simulink model "ansiOctComp"  (R2018a)
settings: Solver=VariableStepAuto  StartTime=0.0  StopTime=0.001  RelTol=1e-3
undefined symbols (not defined in the file): fdesignblkfcn, G1, G2, G3, G4, G5, G6, G7, G8, gcbh, get, T
libraries: dspsrcs4 x1, dspxfrm3 x1, dspobslib x1
(part 3 of 3)

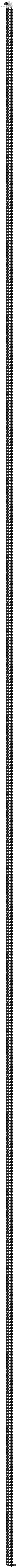
== system ansiOctComp/Filter Bank /Filter 2/Bandpass Filter/Generated Filter Block ==
  Input : Inport
  BodyDelay{2..528} (527 alike) : Delay  DelayLength=1  InitialCondition=0
  BodyLSum{2..528} (527 alike) : Sum  Inputs=++|  RndMeth=Nearest  SaturateOnIntegerOverflow=on  OutDataTypeStr=Inherit: Same as first input
  b(1) : Gain  Gain=0.0013189957886183244  ParamDataTypeStr=double  RndMeth=Nearest  SaturateOnIntegerOverflow=on  OutDataTypeStr=Inherit: Same as input
  b(10) : Gain  Gain=0.000128994813916388394  ParamDataTypeStr=double  RndMeth=Nearest  SaturateOnIntegerOverflow=on  OutDataTypeStr=Inherit: Same as input
  b(100) : Gain  Gain=-0.000423533495409219316  ParamDataTypeStr=double  RndMeth=Nearest  SaturateOnIntegerOverflow=on  OutDataTypeStr=Inherit: Same as input
  b(101) : Gain  Gain=-0.000461669334225578475  ParamDataTypeStr=double  RndMeth=Nearest  SaturateOnIntegerOverflow=on  OutDataTypeStr=Inherit: Same as input
  b(102) : Gain  Gain=-0.000499272274876905349  ParamDataTypeStr=double  RndMeth=Nearest  SaturateOnIntegerOverflow=on  OutDataTypeStr=Inherit: Same as input
  b(103) : Gain  Gain=-0.000536759002049947602  ParamDataTypeStr=double  RndMeth=Nearest  SaturateOnIntegerOverflow=on  OutDataTypeStr=Inherit: Same as input
  b(104) : Gain  Gain=-0.00057288638177031251  ParamDataTypeStr=double  RndMeth=Nearest  SaturateOnIntegerOverflow=on  OutDataTypeStr=Inherit: Same as input
  b(105) : Gain  Gain=-0.000608018296520356112  ParamDataTypeStr=double  RndMeth=Nearest  SaturateOnIntegerOverflow=on  OutDataTypeStr=Inherit: Same as input
  b(106) : Gain  Gain=-0.000640997939764448256  ParamDataTypeStr=double  RndMeth=Nearest  SaturateOnIntegerOverflow=on  OutDataTypeStr=Inherit: Same as input
  b(107) : Gain  Gain=-0.000672143479130331268  ParamDataTypeStr=double  RndMeth=Nearest  SaturateOnIntegerOverflow=on  OutDataTypeStr=Inherit: Same as input
  b(108) : Gain  Gain=-0.000700138237773947664  ParamDataTypeStr=double  RndMeth=Nearest  SaturateOnIntegerOverflow=on  OutDataTypeStr=Inherit: Same as input
  b(109) : Gain  Gain=-0.000725457005707568739  ParamDataTypeStr=double  RndMeth=Nearest  SaturateOnIntegerOverflow=on  OutDataTypeStr=Inherit: Same as input
  b(11) : Gain  Gain=0.000125642526667612978  ParamDataTypeStr=double  RndMeth=Nearest  SaturateOnIntegerOverflow=on  OutDataTypeStr=Inherit: Same as input
  b(110) : Gain  Gain=-0.000746694212294661563  ParamDataTypeStr=double  RndMeth=Nearest  SaturateOnIntegerOverflow=on  OutDataTypeStr=Inherit: Same as input
  b(111) : Gain  Gain=-0.000764284945513389754  ParamDataTypeStr=double  RndMeth=Nearest  SaturateOnIntegerOverflow=on  OutDataTypeStr=Inherit: Same as input
  b(112) : Gain  Gain=-0.000776912328953108179  ParamDataTypeStr=double  RndMeth=Nearest  SaturateOnIntegerOverflow=on  OutDataTypeStr=Inherit: Same as input
  b(113) : Gain  Gain=-0.000784985189046555625  ParamDataTypeStr=double  RndMeth=Nearest  SaturateOnIntegerOverflow=on  OutDataTypeStr=Inherit: Same as input
  b(114) : Gain  Gain=-0.000787233425354552717  ParamDataTypeStr=double  RndMeth=Nearest  SaturateOnIntegerOverflow=on  OutDataTypeStr=Inherit: Same as input
  b(115) : Gain  Gain=-0.00078403753021555095  ParamDataTypeStr=double  RndMeth=Nearest  SaturateOnIntegerOverflow=on  OutDataTypeStr=Inherit: Same as input
  b(116) : Gain  Gain=-0.000774164375811770954  ParamDataTypeStr=double  RndMeth=Nearest  SaturateOnIntegerOverflow=on  OutDataTypeStr=Inherit: Same as input
  b(117) : Gain  Gain=-0.00075805870009854092  ParamDataTypeStr=double  RndMeth=Nearest  SaturateOnIntegerOverflow=on  OutDataTypeStr=Inherit: Same as input
  b(118) : Gain  Gain=-0.000734569828311722726  ParamDataTypeStr=double  RndMeth=Nearest  SaturateOnIntegerOverflow=on  OutDataTypeStr=Inherit: Same as input
  b(119) : Gain  Gain=-0.000704141633403310195  ParamDataTypeStr=double  RndMeth=Nearest  SaturateOnIntegerOverflow=on  OutDataTypeStr=Inherit: Same as input
  b(12) : Gain  Gain=0.000122046249196258033  ParamDataTypeStr=double  RndMeth=Nearest  SaturateOnIntegerOverflow=on  OutDataTypeStr=Inherit: Same as input
  b(120) : Gain  Gain=-0.000665646484304962876  ParamDataTypeStr=double  RndMeth=Nearest  SaturateOnIntegerOverflow=on  OutDataTypeStr=Inherit: Same as input
  b(121) : Gain  Gain=-0.000619640367190464419  ParamDataTypeStr=double  RndMeth=Nearest  SaturateOnIntegerOverflow=on  OutDataTypeStr=Inherit: Same as input
  b(122) : Gain  Gain=-0.000565134472783350244  ParamDataTypeStr=double  RndMeth=Nearest  SaturateOnIntegerOverflow=on  OutDataTypeStr=Inherit: Same as input
  b(123) : Gain  Gain=-0.000502625089221949307  ParamDataTypeStr=double  RndMeth=Nearest  SaturateOnIntegerOverflow=on  OutDataTypeStr=Inherit: Same as input
  b(124) : Gain  Gain=-0.000431307266994649828  ParamDataTypeStr=double  RndMeth=Nearest  SaturateOnIntegerOverflow=on  OutDataTypeStr=Inherit: Same as input
  b(125) : Gain  Gain=-0.000351769691493805832  ParamDataTypeStr=double  RndMeth=Nearest  SaturateOnIntegerOverflow=on  OutDataTypeStr=Inherit: Same as input
  b(126) : Gain  Gain=-0.000263221131644026524  ParamDataTypeStr=double  RndMeth=Nearest  SaturateOnIntegerOverflow=on  OutDataTypeStr=Inherit: Same as input
  b(127) : Gain  Gain=-0.000166409873705706049  ParamDataTypeStr=double  RndMeth=Nearest  SaturateOnIntegerOverflow=on  OutDataTypeStr=Inherit: Same as input
  b(128) : Gain  Gain=-6.06350808818785243e-05  ParamDataTypeStr=double  RndMeth=Nearest  SaturateOnIntegerOverflow=on  OutDataTypeStr=Inherit: Same as input
  b(129) : Gain  Gain=5.3221221105915692e-05  ParamDataTypeStr=double  RndMeth=Nearest  SaturateOnIntegerOverflow=on  OutDataTypeStr=Inherit: Same as input
  b(13) : Gain  Gain=0.000115908705622264248  ParamDataTypeStr=double  RndMeth=Nearest  SaturateOnIntegerOverflow=on  OutDataTypeStr=Inherit: Same as input
  b(130) : Gain  Gain=0.000175769318122429323  ParamDataTypeStr=double  RndMeth=Nearest  SaturateOnIntegerOverflow=on  OutDataTypeStr=Inherit: Same as input
  b(131) : Gain  Gain=0.000306041227612374213  ParamDataTypeStr=double  RndMeth=Nearest  SaturateOnIntegerOverflow=on  OutDataTypeStr=Inherit: Same as input
  b(132) : Gain  Gain=0.000444512367971374497  ParamDataTypeStr=double  RndMeth=Nearest  SaturateOnIntegerOverflow=on  OutDataTypeStr=Inherit: Same as input
  b(133) : Gain  Gain=0.000590057589736560101  ParamDataTypeStr=double  RndMeth=Nearest  SaturateOnIntegerOverflow=on  OutDataTypeStr=Inherit: Same as input
  b(134) : Gain  Gain=0.000743040070891614452  ParamDataTypeStr=double  RndMeth=Nearest  SaturateOnIntegerOverflow=on  OutDataTypeStr=Inherit: Same as input
  b(135) : Gain  Gain=0.000902265678969772192  ParamDataTypeStr=double  RndMeth=Nearest  SaturateOnIntegerOverflow=on  OutDataTypeStr=Inherit: Same as input
  b(136) : Gain  Gain=0.00106797088471714927  ParamDataTypeStr=double  RndMeth=Nearest  SaturateOnIntegerOverflow=on  OutDataTypeStr=Inherit: Same as input
  b(137) : Gain  Gain=0.00123877378306479539  ParamDataTypeStr=double  RndMeth=Nearest  SaturateOnIntegerOverflow=on  OutDataTypeStr=Inherit: Same as input
  b(138) : Gain  Gain=0.00141487218687043554  ParamDataTypeStr=double  RndMeth=Nearest  SaturateOnIntegerOverflow=on  OutDataTypeStr=Inherit: Same as input
  b(139) : Gain  Gain=0.00159476176493942136  ParamDataTypeStr=double  RndMeth=Nearest  SaturateOnIntegerOverflow=on  OutDataTypeStr=Inherit: Same as input
  b(14) : Gain  Gain=0.000109424395758821007  ParamDataTypeStr=double  RndMeth=Nearest  SaturateOnIntegerOverflow=on  OutDataTypeStr=Inherit: Same as input
  b(140) : Gain  Gain=0.00177845198936645564  ParamDataTypeStr=double  RndMeth=Nearest  SaturateOnIntegerOverflow=on  OutDataTypeStr=Inherit: Same as input
  b(141) : Gain  Gain=0.0019644273961855049  ParamDataTypeStr=double  RndMeth=Nearest  SaturateOnIntegerOverflow=on  OutDataTypeStr=Inherit: Same as input
  b(142) : Gain  Gain=0.00215255509300310262  ParamDataTypeStr=double  RndMeth=Nearest  SaturateOnIntegerOverflow=on  OutDataTypeStr=Inherit: Same as input
  b(143) : Gain  Gain=0.00234124102603082635  ParamDataTypeStr=double  RndMeth=Nearest  SaturateOnIntegerOverflow=on  OutDataTypeStr=Inherit: Same as input
  b(144) : Gain  Gain=0.00253023101632903575  ParamDataTypeStr=double  RndMeth=Nearest  SaturateOnIntegerOverflow=on  OutDataTypeStr=Inherit: Same as input
  b(145) : Gain  Gain=0.0027178557454954292  ParamDataTypeStr=double  RndMeth=Nearest  SaturateOnIntegerOverflow=on  OutDataTypeStr=Inherit: Same as input
  b(146) : Gain  Gain=0.00290381159203095124  ParamDataTypeStr=double  RndMeth=Nearest  SaturateOnIntegerOverflow=on  OutDataTypeStr=Inherit: Same as input
  b(147) : Gain  Gain=0.00308638207372412135  ParamDataTypeStr=double  RndMeth=Nearest  SaturateOnIntegerOverflow=on  OutDataTypeStr=Inherit: Same as input
  b(148) : Gain  Gain=0.00326516612697404403  ParamDataTypeStr=double  RndMeth=Nearest  SaturateOnIntegerOverflow=on  OutDataTypeStr=Inherit: Same as input
  b(149) : Gain  Gain=0.00343839387437318202  ParamDataTypeStr=double  RndMeth=Nearest  SaturateOnIntegerOverflow=on  OutDataTypeStr=Inherit: Same as input
  b(15) : Gain  Gain=0.000100118512988072762  ParamDataTypeStr=double  RndMeth=Nearest  SaturateOnIntegerOverflow=on  OutDataTypeStr=Inherit: Same as input
  b(150) : Gain  Gain=0.00360564932851902388  ParamDataTypeStr=double  RndMeth=Nearest  SaturateOnIntegerOverflow=on  OutDataTypeStr=Inherit: Same as input
  b(151) : Gain  Gain=0.00376516794268936172  ParamDataTypeStr=double  RndMeth=Nearest  SaturateOnIntegerOverflow=on  OutDataTypeStr=Inherit: Same as input
  b(152) : Gain  Gain=0.00391645258241414898  ParamDataTypeStr=double  RndMeth=Nearest  SaturateOnIntegerOverflow=on  OutDataTypeStr=Inherit: Same as input
  b(153) : Gain  Gain=0.00405777405273261005  ParamDataTypeStr=double  RndMeth=Nearest  SaturateOnIntegerOverflow=on  OutDataTypeStr=Inherit: Same as input
  b(154) : Gain  Gain=0.00418867978645957092  ParamDataTypeStr=double  RndMeth=Nearest  SaturateOnIntegerOverflow=on  OutDataTypeStr=Inherit: Same as input
  b(155) : Gain  Gain=0.0043073826617828579  ParamDataTypeStr=double  RndMeth=Nearest  SaturateOnIntegerOverflow=on  OutDataTypeStr=Inherit: Same as input
  b(156) : Gain  Gain=0.00441351242527037672  ParamDataTypeStr=double  RndMeth=Nearest  SaturateOnIntegerOverflow=on  OutDataTypeStr=Inherit: Same as input
  b(157) : Gain  Gain=0.00450533688353090857  ParamDataTypeStr=double  RndMeth=Nearest  SaturateOnIntegerOverflow=on  OutDataTypeStr=Inherit: Same as input
  b(158) : Gain  Gain=0.00458254074599091094  ParamDataTypeStr=double  RndMeth=Nearest  SaturateOnIntegerOverflow=on  OutDataTypeStr=Inherit: Same as input
  b(159) : Gain  Gain=0.00464346418155206584  ParamDataTypeStr=double  RndMeth=Nearest  SaturateOnIntegerOverflow=on  OutDataTypeStr=Inherit: Same as input
  b(16) : Gain  Gain=9.42827838523885992e-05  ParamDataTypeStr=double  RndMeth=Nearest  SaturateOnIntegerOverflow=on  OutDataTypeStr=Inherit: Same as input
  b(160) : Gain  Gain=0.00468784260596036978  ParamDataTypeStr=double  RndMeth=Nearest  SaturateOnIntegerOverflow=on  OutDataTypeStr=Inherit: Same as input
  b(161) : Gain  Gain=0.00471414582817185693  ParamDataTypeStr=double  RndMeth=Nearest  SaturateOnIntegerOverflow=on  OutDataTypeStr=Inherit: Same as input
  b(162) : Gain  Gain=0.00472223215326236789  ParamDataTypeStr=double  RndMeth=Nearest  SaturateOnIntegerOverflow=on  OutDataTypeStr=Inherit: Same as input
  b(163) : Gain  Gain=0.00471069265375758696  ParamDataTypeStr=double  RndMeth=Nearest  SaturateOnIntegerOverflow=on  OutDataTypeStr=Inherit: Same as input
  b(164) : Gain  Gain=0.00467948532462431933  ParamDataTypeStr=double  RndMeth=Nearest  SaturateOnIntegerOverflow=on  OutDataTypeStr=Inherit: Same as input
  b(165) : Gain  Gain=0.00462737166796193655  ParamDataTypeStr=double  RndMeth=Nearest  SaturateOnIntegerOverflow=on  OutDataTypeStr=Inherit: Same as input
  b(166) : Gain  Gain=0.00455448397919440591  ParamDataTypeStr=double  RndMeth=Nearest  SaturateOnIntegerOverflow=on  OutDataTypeStr=Inherit: Same as input
  b(167) : Gain  Gain=0.00445973230065942021  ParamDataTypeStr=double  RndMeth=Nearest  SaturateOnIntegerOverflow=on  OutDataTypeStr=Inherit: Same as input
  b(168) : Gain  Gain=0.00434340083942166052  ParamDataTypeStr=double  RndMeth=Nearest  SaturateOnIntegerOverflow=on  OutDataTypeStr=Inherit: Same as input
  b(169) : Gain  Gain=0.00420466577279327014  ParamDataTypeStr=double  RndMeth=Nearest  SaturateOnIntegerOverflow=on  OutDataTypeStr=Inherit: Same as input
  b(17) : Gain  Gain=8.34713962025901597e-05  ParamDataTypeStr=double  RndMeth=Nearest  SaturateOnIntegerOverflow=on  OutDataTypeStr=Inherit: Same as input
  b(170) : Gain  Gain=0.00404392562049606889  ParamDataTypeStr=double  RndMeth=Nearest  SaturateOnIntegerOverflow=on  OutDataTypeStr=Inherit: Same as input
  b(171) : Gain  Gain=0.00386057987620588502  ParamDataTypeStr=double  RndMeth=Nearest  SaturateOnIntegerOverflow=on  OutDataTypeStr=Inherit: Same as input
  b(172) : Gain  Gain=0.00365524307304546667  ParamDataTypeStr=double  RndMeth=Nearest  SaturateOnIntegerOverflow=on  OutDataTypeStr=Inherit: Same as input
  b(173) : Gain  Gain=0.00342754062478000223  ParamDataTypeStr=double  RndMeth=Nearest  SaturateOnIntegerOverflow=on  OutDataTypeStr=Inherit: Same as input
  b(174) : Gain  Gain=0.00317830525562316476  ParamDataTypeStr=double  RndMeth=Nearest  SaturateOnIntegerOverflow=on  OutDataTypeStr=Inherit: Same as input
  b(175) : Gain  Gain=0.00290736343473789721  ParamDataTypeStr=double  RndMeth=Nearest  SaturateOnIntegerOverflow=on  OutDataTypeStr=Inherit: Same as input
  b(176) : Gain  Gain=0.00261576565085099412  ParamDataTypeStr=double  RndMeth=Nearest  SaturateOnIntegerOverflow=on  OutDataTypeStr=Inherit: Same as input
  b(177) : Gain  Gain=0.00230359584321299495  ParamDataTypeStr=double  RndMeth=Nearest  SaturateOnIntegerOverflow=on  OutDataTypeStr=Inherit: Same as input
  b(178) : Gain  Gain=0.00197212374635451606  ParamDataTypeStr=double  RndMeth=Nearest  SaturateOnIntegerOverflow=on  OutDataTypeStr=Inherit: Same as input
  b(179) : Gain  Gain=0.00162164490904748246  ParamDataTypeStr=double  RndMeth=Nearest  SaturateOnIntegerOverflow=on  OutDataTypeStr=Inherit: Same as input
  b(18) : Gain  Gain=7.22562062001517146e-05  ParamDataTypeStr=double  RndMeth=Nearest  SaturateOnIntegerOverflow=on  OutDataTypeStr=Inherit: Same as input
  b(180) : Gain  Gain=0.00125364014383198136  ParamDataTypeStr=double  RndMeth=Nearest  SaturateOnIntegerOverflow=on  OutDataTypeStr=Inherit: Same as input
  b(181) : Gain  Gain=0.000868655989237555122  ParamDataTypeStr=double  RndMeth=Nearest  SaturateOnIntegerOverflow=on  OutDataTypeStr=Inherit: Same as input
  b(182) : Gain  Gain=0.000468370867632063054  ParamDataTypeStr=double  RndMeth=Nearest  SaturateOnIntegerOverflow=on  OutDataTypeStr=Inherit: Same as input
  b(183) : Gain  Gain=5.35140472290680444e-05  ParamDataTypeStr=double  RndMeth=Nearest  SaturateOnIntegerOverflow=on  OutDataTypeStr=Inherit: Same as input
  b(184) : Gain  Gain=-0.000373983290647662229  ParamDataTypeStr=double  RndMeth=Nearest  SaturateOnIntegerOverflow=on  OutDataTypeStr=Inherit: Same as input
  b(185) : Gain  Gain=-0.000813211352745061991  ParamDataTypeStr=double  RndMeth=Nearest  SaturateOnIntegerOverflow=on  OutDataTypeStr=Inherit: Same as input
  b(186) : Gain  Gain=-0.00126209603155125281  ParamDataTypeStr=double  RndMeth=Nearest  SaturateOnIntegerOverflow=on  OutDataTypeStr=Inherit: Same as input
  b(187) : Gain  Gain=-0.0017195185695295912  ParamDataTypeStr=double  RndMeth=Nearest  SaturateOnIntegerOverflow=on  OutDataTypeStr=Inherit: Same as input
  b(188) : Gain  Gain=-0.00218326323704426785  ParamDataTypeStr=double  RndMeth=Nearest  SaturateOnIntegerOverflow=on  OutDataTypeStr=Inherit: Same as input
  b(189) : Gain  Gain=-0.00265202428934371588  ParamDataTypeStr=double  RndMeth=Nearest  SaturateOnIntegerOverflow=on  OutDataTypeStr=Inherit: Same as input
  b(19) : Gain  Gain=6.06151093979667883e-05  ParamDataTypeStr=double  RndMeth=Nearest  SaturateOnIntegerOverflow=on  OutDataTypeStr=Inherit: Same as input
  b(190) : Gain  Gain=-0.00312349066678841922  ParamDataTypeStr=double  RndMeth=Nearest  SaturateOnIntegerOverflow=on  OutDataTypeStr=Inherit: Same as input
  b(191) : Gain  Gain=-0.00359623038932883627  ParamDataTypeStr=double  RndMeth=Nearest  SaturateOnIntegerOverflow=on  OutDataTypeStr=Inherit: Same as input
  b(192) : Gain  Gain=-0.00406783048087909754  ParamDataTypeStr=double  RndMeth=Nearest  SaturateOnIntegerOverflow=on  OutDataTypeStr=Inherit: Same as input
  b(193) : Gain  Gain=-0.00453673939665598207  ParamDataTypeStr=double  RndMeth=Nearest  SaturateOnIntegerOverflow=on  OutDataTypeStr=Inherit: Same as input
  b(194) : Gain  Gain=-0.00500050492305324865  ParamDataTypeStr=double  RndMeth=Nearest  SaturateOnIntegerOverflow=on  OutDataTypeStr=Inherit: Same as input
  b(195) : Gain  Gain=-0.0054575111020349126  ParamDataTypeStr=double  RndMeth=Nearest  SaturateOnIntegerOverflow=on  OutDataTypeStr=Inherit: Same as input
  b(196) : Gain  Gain=-0.00590527600257780439  ParamDataTypeStr=double  RndMeth=Nearest  SaturateOnIntegerOverflow=on  OutDataTypeStr=Inherit: Same as input
  b(197) : Gain  Gain=-0.00634214127357332104  ParamDataTypeStr=double  RndMeth=Nearest  SaturateOnIntegerOverflow=on  OutDataTypeStr=Inherit: Same as input
  b(198) : Gain  Gain=-0.00676568738089359037  ParamDataTypeStr=double  RndMeth=Nearest  SaturateOnIntegerOverflow=on  OutDataTypeStr=Inherit: Same as input
  b(199) : Gain  Gain=-0.00717422804624558326  ParamDataTypeStr=double  RndMeth=Nearest  SaturateOnIntegerOverflow=on  OutDataTypeStr=Inherit: Same as input
  b(2) : Gain  Gain=0.000119600445182501628  ParamDataTypeStr=double  RndMeth=Nearest  SaturateOnIntegerOverflow=on  OutDataTypeStr=Inherit: Same as input
  b(20) : Gain  Gain=4.75559208421214279e-05  ParamDataTypeStr=double  RndMeth=Nearest  SaturateOnIntegerOverflow=on  OutDataTypeStr=Inherit: Same as input
  b(200) : Gain  Gain=-0.00756538283354352657  ParamDataTypeStr=double  RndMeth=Nearest  SaturateOnIntegerOverflow=on  OutDataTypeStr=Inherit: Same as input
  b(201) : Gain  Gain=-0.00793755453304027976  ParamDataTypeStr=double  RndMeth=Nearest  SaturateOnIntegerOverflow=on  OutDataTypeStr=Inherit: Same as input
  b(202) : Gain  Gain=-0.00828844414503448167  ParamDataTypeStr=double  RndMeth=Nearest  SaturateOnIntegerOverflow=on  OutDataTypeStr=Inherit: Same as input
  b(203) : Gain  Gain=-0.00861655179384803772  ParamDataTypeStr=double  RndMeth=Nearest  SaturateOnIntegerOverflow=on  OutDataTypeStr=Inherit: Same as input
  b(204) : Gain  Gain=-0.00891968858251965604  ParamDataTypeStr=double  RndMeth=Nearest  SaturateOnIntegerOverflow=on  OutDataTypeStr=Inherit: Same as input
  b(205) : Gain  Gain=-0.00919649068666273176  ParamDataTypeStr=double  RndMeth=Nearest  SaturateOnIntegerOverflow=on  OutDataTypeStr=Inherit: Same as input
  b(206) : Gain  Gain=-0.00944496004746541058  ParamDataTypeStr=double  RndMeth=Nearest  SaturateOnIntegerOverflow=on  OutDataTypeStr=Inherit: Same as input
  b(207) : Gain  Gain=-0.00966389591080612023  ParamDataTypeStr=double  RndMeth=Nearest  SaturateOnIntegerOverflow=on  OutDataTypeStr=Inherit: Same as input
  b(208) : Gain  Gain=-0.0098514944054812776  ParamDataTypeStr=double  RndMeth=Nearest  SaturateOnIntegerOverflow=on  OutDataTypeStr=Inherit: Same as input
  b(209) : Gain  Gain=-0.010006763264188796  ParamDataTypeStr=double  RndMeth=Nearest  SaturateOnIntegerOverflow=on  OutDataTypeStr=Inherit: Same as input
  b(21) : Gain  Gain=3.35500754738617818e-05  ParamDataTypeStr=double  RndMeth=Nearest  SaturateOnIntegerOverflow=on  OutDataTypeStr=Inherit: Same as input
  b(210) : Gain  Gain=-0.0101281486721101384  ParamDataTypeStr=double  RndMeth=Nearest  SaturateOnIntegerOverflow=on  OutDataTypeStr=Inherit: Same as input
  b(211) : Gain  Gain=-0.0102148848795295486  ParamDataTypeStr=double  RndMeth=Nearest  SaturateOnIntegerOverflow=on  OutDataTypeStr=Inherit: Same as input
  b(212) : Gain  Gain=-0.0102656745807170411  ParamDataTypeStr=double  RndMeth=Nearest  SaturateOnIntegerOverflow=on  OutDataTypeStr=Inherit: Same as input
  b(213) : Gain  Gain=-0.0102800430916763635  ParamDataTypeStr=double  RndMeth=Nearest  SaturateOnIntegerOverflow=on  OutDataTypeStr=Inherit: Same as input
  b(214) : Gain  Gain=-0.0102569951229774387  ParamDataTypeStr=double  RndMeth=Nearest  SaturateOnIntegerOverflow=on  OutDataTypeStr=Inherit: Same as input
  b(215) : Gain  Gain=-0.0101962935444855421  ParamDataTypeStr=double  RndMeth=Nearest  SaturateOnIntegerOverflow=on  OutDataTypeStr=Inherit: Same as input
  b(216) : Gain  Gain=-0.0100972980487470266  ParamDataTypeStr=double  RndMeth=Nearest  SaturateOnIntegerOverflow=on  OutDataTypeStr=Inherit: Same as input
  b(217) : Gain  Gain=-0.00996006829043967305  ParamDataTypeStr=double  RndMeth=Nearest  SaturateOnIntegerOverflow=on  OutDataTypeStr=Inherit: Same as input
  b(218) : Gain  Gain=-0.00978431184645446768  ParamDataTypeStr=double  RndMeth=Nearest  SaturateOnIntegerOverflow=on  OutDataTypeStr=Inherit: Same as input
  b(219) : Gain  Gain=-0.00957038326330438699  ParamDataTypeStr=double  RndMeth=Nearest  SaturateOnIntegerOverflow=on  OutDataTypeStr=Inherit: Same as input
  b(22) : Gain  Gain=1.85707383679374095e-05  ParamDataTypeStr=double  RndMeth=Nearest  SaturateOnIntegerOverflow=on  OutDataTypeStr=Inherit: Same as input
  b(220) : Gain  Gain=-0.00931832776697521722  ParamDataTypeStr=double  RndMeth=Nearest  SaturateOnIntegerOverflow=on  OutDataTypeStr=Inherit: Same as input
  b(221) : Gain  Gain=-0.00902883400440002842  ParamDataTypeStr=double  RndMeth=Nearest  SaturateOnIntegerOverflow=on  OutDataTypeStr=Inherit: Same as input
  b(222) : Gain  Gain=-0.0087022994301005855  ParamDataTypeStr=double  RndMeth=Nearest  SaturateOnIntegerOverflow=on  OutDataTypeStr=Inherit: Same as input
  b(223) : Gain  Gain=-0.00833971895740222291  ParamDataTypeStr=double  RndMeth=Nearest  SaturateOnIntegerOverflow=on  OutDataTypeStr=Inherit: Same as input
  b(224) : Gain  Gain=-0.00794183669351568484  ParamDataTypeStr=double  RndMeth=Nearest  SaturateOnIntegerOverflow=on  OutDataTypeStr=Inherit: Same as input
  b(225) : Gain  Gain=-0.0075099688685431789  ParamDataTypeStr=double  RndMeth=Nearest  SaturateOnIntegerOverflow=on  OutDataTypeStr=Inherit: Same as input
  b(226) : Gain  Gain=-0.00704519052646493914  ParamDataTypeStr=double  RndMeth=Nearest  SaturateOnIntegerOverflow=on  OutDataTypeStr=Inherit: Same as input
  b(227) : Gain  Gain=-0.00654910227540862235  ParamDataTypeStr=double  RndMeth=Nearest  SaturateOnIntegerOverflow=on  OutDataTypeStr=Inherit: Same as input
  b(228) : Gain  Gain=-0.00602310593375914981  ParamDataTypeStr=double  RndMeth=Nearest  SaturateOnIntegerOverflow=on  OutDataTypeStr=Inherit: Same as input
  b(229) : Gain  Gain=-0.00546911525876405454  ParamDataTypeStr=double  RndMeth=Nearest  SaturateOnIntegerOverflow=on  OutDataTypeStr=Inherit: Same as input
  b(23) : Gain  Gain=2.53229324894679517e-06  ParamDataTypeStr=double  RndMeth=Nearest  SaturateOnIntegerOverflow=on  OutDataTypeStr=Inherit: Same as input
  b(230) : Gain  Gain=-0.00488877924777270882  ParamDataTypeStr=double  RndMeth=Nearest  SaturateOnIntegerOverflow=on  OutDataTypeStr=Inherit: Same as input
  b(231) : Gain  Gain=-0.00428427881908863967  ParamDataTypeStr=double  RndMeth=Nearest  SaturateOnIntegerOverflow=on  OutDataTypeStr=Inherit: Same as input
  b(232) : Gain  Gain=-0.00365753396240067925  ParamDataTypeStr=double  RndMeth=Nearest  SaturateOnIntegerOverflow=on  OutDataTypeStr=Inherit: Same as input
  b(233) : Gain  Gain=-0.00301096103934305002  ParamDataTypeStr=double  RndMeth=Nearest  SaturateOnIntegerOverflow=on  OutDataTypeStr=Inherit: Same as input
  b(234) : Gain  Gain=-0.00234670804643675145  ParamDataTypeStr=double  RndMeth=Nearest  SaturateOnIntegerOverflow=on  OutDataTypeStr=Inherit: Same as input
  b(235) : Gain  Gain=-0.0016673640491828871  ParamDataTypeStr=double  RndMeth=Nearest  SaturateOnIntegerOverflow=on  OutDataTypeStr=Inherit: Same as input
  b(236) : Gain  Gain=-0.000975280953428218672  ParamDataTypeStr=double  RndMeth=Nearest  SaturateOnIntegerOverflow=on  OutDataTypeStr=Inherit: Same as input
  b(237) : Gain  Gain=-0.000273203447335550621  ParamDataTypeStr=double  RndMeth=Nearest  SaturateOnIntegerOverflow=on  OutDataTypeStr=Inherit: Same as input
  b(238) : Gain  Gain=0.000436374222012142076  ParamDataTypeStr=double  RndMeth=Nearest  SaturateOnIntegerOverflow=on  OutDataTypeStr=Inherit: Same as input
  b(239) : Gain  Gain=0.00115060614139325798  ParamDataTypeStr=double  RndMeth=Nearest  SaturateOnIntegerOverflow=on  OutDataTypeStr=Inherit: Same as input
  b(24) : Gain  Gain=-1.41991623558972851e-05  ParamDataTypeStr=double  RndMeth=Nearest  SaturateOnIntegerOverflow=on  OutDataTypeStr=Inherit: Same as input
  b(240) : Gain  Gain=0.00186688192354099339  ParamDataTypeStr=double  RndMeth=Nearest  SaturateOnIntegerOverflow=on  OutDataTypeStr=Inherit: Same as input
  b(241) : Gain  Gain=0.0025823010557774642  ParamDataTypeStr=double  RndMeth=Nearest  SaturateOnIntegerOverflow=on  OutDataTypeStr=Inherit: Same as input
  b(242) : Gain  Gain=0.00329420582374038984  ParamDataTypeStr=double  RndMeth=Nearest  SaturateOnIntegerOverflow=on  OutDataTypeStr=Inherit: Same as input
  b(243) : Gain  Gain=0.0039996992447598927  ParamDataTypeStr=double  RndMeth=Nearest  SaturateOnIntegerOverflow=on  OutDataTypeStr=Inherit: Same as input
  b(244) : Gain  Gain=0.00469607268691952899  ParamDataTypeStr=double  RndMeth=Nearest  SaturateOnIntegerOverflow=on  OutDataTypeStr=Inherit: Same as input
  b(245) : Gain  Gain=0.0053804949397835691  ParamDataTypeStr=double  RndMeth=Nearest  SaturateOnIntegerOverflow=on  OutDataTypeStr=Inherit: Same as input
  b(246) : Gain  Gain=0.00605031412425023618  ParamDataTypeStr=double  RndMeth=Nearest  SaturateOnIntegerOverflow=on  OutDataTypeStr=Inherit: Same as input
  b(247) : Gain  Gain=0.00670277986405692482  ParamDataTypeStr=double  RndMeth=Nearest  SaturateOnIntegerOverflow=on  OutDataTypeStr=Inherit: Same as input
  b(248) : Gain  Gain=0.00733532884864761432  ParamDataTypeStr=double  RndMeth=Nearest  SaturateOnIntegerOverflow=on  OutDataTypeStr=Inherit: Same as input
  b(249) : Gain  Gain=0.00794534100781414503  ParamDataTypeStr=double  RndMeth=Nearest  SaturateOnIntegerOverflow=on  OutDataTypeStr=Inherit: Same as input
  b(25) : Gain  Gain=-3.18260172032644104e-05  ParamDataTypeStr=double  RndMeth=Nearest  SaturateOnIntegerOverflow=on  OutDataTypeStr=Inherit: Same as input
  b(250) : Gain  Gain=0.00853041422830583609  ParamDataTypeStr=double  RndMeth=Nearest  SaturateOnIntegerOverflow=on  OutDataTypeStr=Inherit: Same as input
  b(251) : Gain  Gain=0.00908810793177476477  ParamDataTypeStr=double  RndMeth=Nearest  SaturateOnIntegerOverflow=on  OutDataTypeStr=Inherit: Same as input
  b(252) : Gain  Gain=0.0096162011798594238  ParamDataTypeStr=double  RndMeth=Nearest  SaturateOnIntegerOverflow=on  OutDataTypeStr=Inherit: Same as input
  b(253) : Gain  Gain=0.0101124848863965184  ParamDataTypeStr=double  RndMeth=Nearest  SaturateOnIntegerOverflow=on  OutDataTypeStr=Inherit: Same as input
  b(254) : Gain  Gain=0.010574977470715138  ParamDataTypeStr=double  RndMeth=Nearest  SaturateOnIntegerOverflow=on  OutDataTypeStr=Inherit: Same as input
  b(255) : Gain  Gain=0.0110017227247066317  ParamDataTypeStr=double  RndMeth=Nearest  SaturateOnIntegerOverflow=on  OutDataTypeStr=Inherit: Same as input
  b(256) : Gain  Gain=0.0113910099520570553  ParamDataTypeStr=double  RndMeth=Nearest  SaturateOnIntegerOverflow=on  OutDataTypeStr=Inherit: Same as input
  b(257) : Gain  Gain=0.0117411869510578616  ParamDataTypeStr=double  RndMeth=Nearest  SaturateOnIntegerOverflow=on  OutDataTypeStr=Inherit: Same as input
  b(258) : Gain  Gain=0.0120508720478830142  ParamDataTypeStr=double  RndMeth=Nearest  SaturateOnIntegerOverflow=on  OutDataTypeStr=Inherit: Same as input
  b(259) : Gain  Gain=0.0123187129332444495  ParamDataTypeStr=double  RndMeth=Nearest  SaturateOnIntegerOverflow=on  OutDataTypeStr=Inherit: Same as input
  b(26) : Gain  Gain=-4.98086298525179418e-05  ParamDataTypeStr=double  RndMeth=Nearest  SaturateOnIntegerOverflow=on  OutDataTypeStr=Inherit: Same as input
  b(260) : Gain  Gain=0.012543649889335623  ParamDataTypeStr=double  RndMeth=Nearest  SaturateOnIntegerOverflow=on  OutDataTypeStr=Inherit: Same as input
  b(261) : Gain  Gain=0.0127247157071038938  ParamDataTypeStr=double  RndMeth=Nearest  SaturateOnIntegerOverflow=on  OutDataTypeStr=Inherit: Same as input
  b(262) : Gain  Gain=0.0128611926097951038  ParamDataTypeStr=double  RndMeth=Nearest  SaturateOnIntegerOverflow=on  OutDataTypeStr=Inherit: Same as input
  b(263) : Gain  Gain=0.0129524876225628471  ParamDataTypeStr=double  RndMeth=Nearest  SaturateOnIntegerOverflow=on  OutDataTypeStr=Inherit: Same as input
  b(264) : Gain  Gain=0.0129982310171642586  ParamDataTypeStr=double  RndMeth=Nearest  SaturateOnIntegerOverflow=on  OutDataTypeStr=Inherit: Same as input
  b(265) : Gain  Gain=0.0129982310171642586  ParamDataTypeStr=double  RndMeth=Nearest  SaturateOnIntegerOverflow=on  OutDataTypeStr=Inherit: Same as input
  b(266) : Gain  Gain=0.0129524876225628471  ParamDataTypeStr=double  RndMeth=Nearest  SaturateOnIntegerOverflow=on  OutDataTypeStr=Inherit: Same as input
  b(267) : Gain  Gain=0.0128611926097951038  ParamDataTypeStr=double  RndMeth=Nearest  SaturateOnIntegerOverflow=on  OutDataTypeStr=Inherit: Same as input
  b(268) : Gain  Gain=0.0127247157071038938  ParamDataTypeStr=double  RndMeth=Nearest  SaturateOnIntegerOverflow=on  OutDataTypeStr=Inherit: Same as input
  b(269) : Gain  Gain=0.012543649889335623  ParamDataTypeStr=double  RndMeth=Nearest  SaturateOnIntegerOverflow=on  OutDataTypeStr=Inherit: Same as input
  b(27) : Gain  Gain=-6.84426124636459271e-05  ParamDataTypeStr=double  RndMeth=Nearest  SaturateOnIntegerOverflow=on  OutDataTypeStr=Inherit: Same as input
  b(270) : Gain  Gain=0.0123187129332444495  ParamDataTypeStr=double  RndMeth=Nearest  SaturateOnIntegerOverflow=on  OutDataTypeStr=Inherit: Same as input
  b(271) : Gain  Gain=0.0120508720478830142  ParamDataTypeStr=double  RndMeth=Nearest  SaturateOnIntegerOverflow=on  OutDataTypeStr=Inherit: Same as input
  b(272) : Gain  Gain=0.0117411869510578616  ParamDataTypeStr=double  RndMeth=Nearest  SaturateOnIntegerOverflow=on  OutDataTypeStr=Inherit: Same as input
  b(273) : Gain  Gain=0.0113910099520570553  ParamDataTypeStr=double  RndMeth=Nearest  SaturateOnIntegerOverflow=on  OutDataTypeStr=Inherit: Same as input
  b(274) : Gain  Gain=0.0110017227247066317  ParamDataTypeStr=double  RndMeth=Nearest  SaturateOnIntegerOverflow=on  OutDataTypeStr=Inherit: Same as input
  b(275) : Gain  Gain=0.010574977470715138  ParamDataTypeStr=double  RndMeth=Nearest  SaturateOnIntegerOverflow=on  OutDataTypeStr=Inherit: Same as input
  b(276) : Gain  Gain=0.0101124848863965184  ParamDataTypeStr=double  RndMeth=Nearest  SaturateOnIntegerOverflow=on  OutDataTypeStr=Inherit: Same as input
  b(277) : Gain  Gain=0.0096162011798594238  ParamDataTypeStr=double  RndMeth=Nearest  SaturateOnIntegerOverflow=on  OutDataTypeStr=Inherit: Same as input
  b(278) : Gain  Gain=0.00908810793177476477  ParamDataTypeStr=double  RndMeth=Nearest  SaturateOnIntegerOverflow=on  OutDataTypeStr=Inherit: Same as input
  b(279) : Gain  Gain=0.00853041422830583609  ParamDataTypeStr=double  RndMeth=Nearest  SaturateOnIntegerOverflow=on  OutDataTypeStr=Inherit: Same as input
  b(28) : Gain  Gain=-8.73504816807577078e-05  ParamDataTypeStr=double  RndMeth=Nearest  SaturateOnIntegerOverflow=on  OutDataTypeStr=Inherit: Same as input
  b(280) : Gain  Gain=0.00794534100781414503  ParamDataTypeStr=double  RndMeth=Nearest  SaturateOnIntegerOverflow=on  OutDataTypeStr=Inherit: Same as input
  b(281) : Gain  Gain=0.00733532884864761432  ParamDataTypeStr=double  RndMeth=Nearest  SaturateOnIntegerOverflow=on  OutDataTypeStr=Inherit: Same as input
  b(282) : Gain  Gain=0.00670277986405692482  ParamDataTypeStr=double  RndMeth=Nearest  SaturateOnIntegerOverflow=on  OutDataTypeStr=Inherit: Same as input
  b(283) : Gain  Gain=0.00605031412425023618  ParamDataTypeStr=double  RndMeth=Nearest  SaturateOnIntegerOverflow=on  OutDataTypeStr=Inherit: Same as input
  b(284) : Gain  Gain=0.0053804949397835691  ParamDataTypeStr=double  RndMeth=Nearest  SaturateOnIntegerOverflow=on  OutDataTypeStr=Inherit: Same as input
  b(285) : Gain  Gain=0.00469607268691952899  ParamDataTypeStr=double  RndMeth=Nearest  SaturateOnIntegerOverflow=on  OutDataTypeStr=Inherit: Same as input
  b(286) : Gain  Gain=0.0039996992447598927  ParamDataTypeStr=double  RndMeth=Nearest  SaturateOnIntegerOverflow=on  OutDataTypeStr=Inherit: Same as input
  b(287) : Gain  Gain=0.00329420582374038984  ParamDataTypeStr=double  RndMeth=Nearest  SaturateOnIntegerOverflow=on  OutDataTypeStr=Inherit: Same as input
  b(288) : Gain  Gain=0.0025823010557774642  ParamDataTypeStr=double  RndMeth=Nearest  SaturateOnIntegerOverflow=on  OutDataTypeStr=Inherit: Same as input
  b(289) : Gain  Gain=0.00186688192354099339  ParamDataTypeStr=double  RndMeth=Nearest  SaturateOnIntegerOverflow=on  OutDataTypeStr=Inherit: Same as input
  b(29) : Gain  Gain=-0.000106978433770536828  ParamDataTypeStr=double  RndMeth=Nearest  SaturateOnIntegerOverflow=on  OutDataTypeStr=Inherit: Same as input
  b(290) : Gain  Gain=0.00115060614139325798  ParamDataTypeStr=double  RndMeth=Nearest  SaturateOnIntegerOverflow=on  OutDataTypeStr=Inherit: Same as input
  b(291) : Gain  Gain=0.000436374222012142076  ParamDataTypeStr=double  RndMeth=Nearest  SaturateOnIntegerOverflow=on  OutDataTypeStr=Inherit: Same as input
  b(292) : Gain  Gain=-0.000273203447335550621  ParamDataTypeStr=double  RndMeth=Nearest  SaturateOnIntegerOverflow=on  OutDataTypeStr=Inherit: Same as input
  b(293) : Gain  Gain=-0.000975280953428218672  ParamDataTypeStr=double  RndMeth=Nearest  SaturateOnIntegerOverflow=on  OutDataTypeStr=Inherit: Same as input
  b(294) : Gain  Gain=-0.0016673640491828871  ParamDataTypeStr=double  RndMeth=Nearest  SaturateOnIntegerOverflow=on  OutDataTypeStr=Inherit: Same as input
  b(295) : Gain  Gain=-0.00234670804643675145  ParamDataTypeStr=double  RndMeth=Nearest  SaturateOnIntegerOverflow=on  OutDataTypeStr=Inherit: Same as input
  b(296) : Gain  Gain=-0.00301096103934305002  ParamDataTypeStr=double  RndMeth=Nearest  SaturateOnIntegerOverflow=on  OutDataTypeStr=Inherit: Same as input
  b(297) : Gain  Gain=-0.00365753396240067925  ParamDataTypeStr=double  RndMeth=Nearest  SaturateOnIntegerOverflow=on  OutDataTypeStr=Inherit: Same as input
  b(298) : Gain  Gain=-0.00428427881908863967  ParamDataTypeStr=double  RndMeth=Nearest  SaturateOnIntegerOverflow=on  OutDataTypeStr=Inherit: Same as input
  b(299) : Gain  Gain=-0.00488877924777270882  ParamDataTypeStr=double  RndMeth=Nearest  SaturateOnIntegerOverflow=on  OutDataTypeStr=Inherit: Same as input
  b(3) : Gain  Gain=0.000123292979075959085  ParamDataTypeStr=double  RndMeth=Nearest  SaturateOnIntegerOverflow=on  OutDataTypeStr=Inherit: Same as input
  b(30) : Gain  Gain=-0.000127069818868432967  ParamDataTypeStr=double  RndMeth=Nearest  SaturateOnIntegerOverflow=on  OutDataTypeStr=Inherit: Same as input
  b(300) : Gain  Gain=-0.00546911525876405454  ParamDataTypeStr=double  RndMeth=Nearest  SaturateOnIntegerOverflow=on  OutDataTypeStr=Inherit: Same as input
  b(301) : Gain  Gain=-0.00602310593375914981  ParamDataTypeStr=double  RndMeth=Nearest  SaturateOnIntegerOverflow=on  OutDataTypeStr=Inherit: Same as input
  b(302) : Gain  Gain=-0.00654910227540862235  ParamDataTypeStr=double  RndMeth=Nearest  SaturateOnIntegerOverflow=on  OutDataTypeStr=Inherit: Same as input
  b(303) : Gain  Gain=-0.00704519052646493914  ParamDataTypeStr=double  RndMeth=Nearest  SaturateOnIntegerOverflow=on  OutDataTypeStr=Inherit: Same as input
  b(304) : Gain  Gain=-0.0075099688685431789  ParamDataTypeStr=double  RndMeth=Nearest  SaturateOnIntegerOverflow=on  OutDataTypeStr=Inherit: Same as input
  b(305) : Gain  Gain=-0.00794183669351568484  ParamDataTypeStr=double  RndMeth=Nearest  SaturateOnIntegerOverflow=on  OutDataTypeStr=Inherit: Same as input
  b(306) : Gain  Gain=-0.00833971895740222291  ParamDataTypeStr=double  RndMeth=Nearest  SaturateOnIntegerOverflow=on  OutDataTypeStr=Inherit: Same as input
  b(307) : Gain  Gain=-0.0087022994301005855  ParamDataTypeStr=double  RndMeth=Nearest  SaturateOnIntegerOverflow=on  OutDataTypeStr=Inherit: Same as input
  b(308) : Gain  Gain=-0.00902883400440002842  ParamDataTypeStr=double  RndMeth=Nearest  SaturateOnIntegerOverflow=on  OutDataTypeStr=Inherit: Same as input
  b(309) : Gain  Gain=-0.00931832776697521722  ParamDataTypeStr=double  RndMeth=Nearest  SaturateOnIntegerOverflow=on  OutDataTypeStr=Inherit: Same as input
  b(31) : Gain  Gain=-0.000146832212862152119  ParamDataTypeStr=double  RndMeth=Nearest  SaturateOnIntegerOverflow=on  OutDataTypeStr=Inherit: Same as input
  b(310) : Gain  Gain=-0.00957038326330438699  ParamDataTypeStr=double  RndMeth=Nearest  SaturateOnIntegerOverflow=on  OutDataTypeStr=Inherit: Same as input
  b(311) : Gain  Gain=-0.00978431184645446768  ParamDataTypeStr=double  RndMeth=Nearest  SaturateOnIntegerOverflow=on  OutDataTypeStr=Inherit: Same as input
  b(312) : Gain  Gain=-0.00996006829043967305  ParamDataTypeStr=double  RndMeth=Nearest  SaturateOnIntegerOverflow=on  OutDataTypeStr=Inherit: Same as input
  b(313) : Gain  Gain=-0.0100972980487470266  ParamDataTypeStr=double  RndMeth=Nearest  SaturateOnIntegerOverflow=on  OutDataTypeStr=Inherit: Same as input
  b(314) : Gain  Gain=-0.0101962935444855421  ParamDataTypeStr=double  RndMeth=Nearest  SaturateOnIntegerOverflow=on  OutDataTypeStr=Inherit: Same as input
  b(315) : Gain  Gain=-0.0102569951229774387  ParamDataTypeStr=double  RndMeth=Nearest  SaturateOnIntegerOverflow=on  OutDataTypeStr=Inherit: Same as input
  b(316) : Gain  Gain=-0.0102800430916763635  ParamDataTypeStr=double  RndMeth=Nearest  SaturateOnIntegerOverflow=on  OutDataTypeStr=Inherit: Same as input
  b(317) : Gain  Gain=-0.0102656745807170411  ParamDataTypeStr=double  RndMeth=Nearest  SaturateOnIntegerOverflow=on  OutDataTypeStr=Inherit: Same as input
  b(318) : Gain  Gain=-0.0102148848795295486  ParamDataTypeStr=double  RndMeth=Nearest  SaturateOnIntegerOverflow=on  OutDataTypeStr=Inherit: Same as input
  b(319) : Gain  Gain=-0.0101281486721101384  ParamDataTypeStr=double  RndMeth=Nearest  SaturateOnIntegerOverflow=on  OutDataTypeStr=Inherit: Same as input
  b(32) : Gain  Gain=-0.000166417949659631399  ParamDataTypeStr=double  RndMeth=Nearest  SaturateOnIntegerOverflow=on  OutDataTypeStr=Inherit: Same as input
  b(320) : Gain  Gain=-0.010006763264188796  ParamDataTypeStr=double  RndMeth=Nearest  SaturateOnIntegerOverflow=on  OutDataTypeStr=Inherit: Same as input
  b(321) : Gain  Gain=-0.0098514944054812776  ParamDataTypeStr=double  RndMeth=Nearest  SaturateOnIntegerOverflow=on  OutDataTypeStr=Inherit: Same as input
  b(322) : Gain  Gain=-0.00966389591080612023  ParamDataTypeStr=double  RndMeth=Nearest  SaturateOnIntegerOverflow=on  OutDataTypeStr=Inherit: Same as input
  b(323) : Gain  Gain=-0.00944496004746541058  ParamDataTypeStr=double  RndMeth=Nearest  SaturateOnIntegerOverflow=on  OutDataTypeStr=Inherit: Same as input
  b(324) : Gain  Gain=-0.00919649068666273176  ParamDataTypeStr=double  RndMeth=Nearest  SaturateOnIntegerOverflow=on  OutDataTypeStr=Inherit: Same as input
  b(325) : Gain  Gain=-0.00891968858251965604  ParamDataTypeStr=double  RndMeth=Nearest  SaturateOnIntegerOverflow=on  OutDataTypeStr=Inherit: Same as input
  b(326) : Gain  Gain=-0.00861655179384803772  ParamDataTypeStr=double  RndMeth=Nearest  SaturateOnIntegerOverflow=on  OutDataTypeStr=Inherit: Same as input
  b(327) : Gain  Gain=-0.00828844414503448167  ParamDataTypeStr=double  RndMeth=Nearest  SaturateOnIntegerOverflow=on  OutDataTypeStr=Inherit: Same as input
  b(328) : Gain  Gain=-0.00793755453304027976  ParamDataTypeStr=double  RndMeth=Nearest  SaturateOnIntegerOverflow=on  OutDataTypeStr=Inherit: Same as input
  b(329) : Gain  Gain=-0.00756538283354352657  ParamDataTypeStr=double  RndMeth=Nearest  SaturateOnIntegerOverflow=on  OutDataTypeStr=Inherit: Same as input
  b(33) : Gain  Gain=-0.000186903105556324297  ParamDataTypeStr=double  RndMeth=Nearest  SaturateOnIntegerOverflow=on  OutDataTypeStr=Inherit: Same as input
  b(330) : Gain  Gain=-0.00717422804624558326  ParamDataTypeStr=double  RndMeth=Nearest  SaturateOnIntegerOverflow=on  OutDataTypeStr=Inherit: Same as input
  b(331) : Gain  Gain=-0.00676568738089359037  ParamDataTypeStr=double  RndMeth=Nearest  SaturateOnIntegerOverflow=on  OutDataTypeStr=Inherit: Same as input
  b(332) : Gain  Gain=-0.00634214127357332104  ParamDataTypeStr=double  RndMeth=Nearest  SaturateOnIntegerOverflow=on  OutDataTypeStr=Inherit: Same as input
  b(333) : Gain  Gain=-0.00590527600257780439  ParamDataTypeStr=double  RndMeth=Nearest  SaturateOnIntegerOverflow=on  OutDataTypeStr=Inherit: Same as input
  b(334) : Gain  Gain=-0.0054575111020349126  ParamDataTypeStr=double  RndMeth=Nearest  SaturateOnIntegerOverflow=on  OutDataTypeStr=Inherit: Same as input
  b(335) : Gain  Gain=-0.00500050492305324865  ParamDataTypeStr=double  RndMeth=Nearest  SaturateOnIntegerOverflow=on  OutDataTypeStr=Inherit: Same as input
  b(336) : Gain  Gain=-0.00453673939665598207  ParamDataTypeStr=double  RndMeth=Nearest  SaturateOnIntegerOverflow=on  OutDataTypeStr=Inherit: Same as input
  b(337) : Gain  Gain=-0.00406783048087909754  ParamDataTypeStr=double  RndMeth=Nearest  SaturateOnIntegerOverflow=on  OutDataTypeStr=Inherit: Same as input
  b(338) : Gain  Gain=-0.00359623038932883627  ParamDataTypeStr=double  RndMeth=Nearest  SaturateOnIntegerOverflow=on  OutDataTypeStr=Inherit: Same as input
  b(339) : Gain  Gain=-0.00312349066678841922  ParamDataTypeStr=double  RndMeth=Nearest  SaturateOnIntegerOverflow=on  OutDataTypeStr=Inherit: Same as input
  b(34) : Gain  Gain=-0.000206139072550225958  ParamDataTypeStr=double  RndMeth=Nearest  SaturateOnIntegerOverflow=on  OutDataTypeStr=Inherit: Same as input
  b(340) : Gain  Gain=-0.00265202428934371588  ParamDataTypeStr=double  RndMeth=Nearest  SaturateOnIntegerOverflow=on  OutDataTypeStr=Inherit: Same as input
  b(341) : Gain  Gain=-0.00218326323704426785  ParamDataTypeStr=double  RndMeth=Nearest  SaturateOnIntegerOverflow=on  OutDataTypeStr=Inherit: Same as input
  b(342) : Gain  Gain=-0.0017195185695295912  ParamDataTypeStr=double  RndMeth=Nearest  SaturateOnIntegerOverflow=on  OutDataTypeStr=Inherit: Same as input
  b(343) : Gain  Gain=-0.00126209603155125281  ParamDataTypeStr=double  RndMeth=Nearest  SaturateOnIntegerOverflow=on  OutDataTypeStr=Inherit: Same as input
  b(344) : Gain  Gain=-0.000813211352745061991  ParamDataTypeStr=double  RndMeth=Nearest  SaturateOnIntegerOverflow=on  OutDataTypeStr=Inherit: Same as input
  b(345) : Gain  Gain=-0.000373983290647662229  ParamDataTypeStr=double  RndMeth=Nearest  SaturateOnIntegerOverflow=on  OutDataTypeStr=Inherit: Same as input
  b(346) : Gain  Gain=5.35140472290680444e-05  ParamDataTypeStr=double  RndMeth=Nearest  SaturateOnIntegerOverflow=on  OutDataTypeStr=Inherit: Same as input
  b(347) : Gain  Gain=0.000468370867632063054  ParamDataTypeStr=double  RndMeth=Nearest  SaturateOnIntegerOverflow=on  OutDataTypeStr=Inherit: Same as input
  b(348) : Gain  Gain=0.000868655989237555122  ParamDataTypeStr=double  RndMeth=Nearest  SaturateOnIntegerOverflow=on  OutDataTypeStr=Inherit: Same as input
  b(349) : Gain  Gain=0.00125364014383198136  ParamDataTypeStr=double  RndMeth=Nearest  SaturateOnIntegerOverflow=on  OutDataTypeStr=Inherit: Same as input
  b(35) : Gain  Gain=-0.000225875280666558518  ParamDataTypeStr=double  RndMeth=Nearest  SaturateOnIntegerOverflow=on  OutDataTypeStr=Inherit: Same as input
  b(350) : Gain  Gain=0.00162164490904748246  ParamDataTypeStr=double  RndMeth=Nearest  SaturateOnIntegerOverflow=on  OutDataTypeStr=Inherit: Same as input
  b(351) : Gain  Gain=0.00197212374635451606  ParamDataTypeStr=double  RndMeth=Nearest  SaturateOnIntegerOverflow=on  OutDataTypeStr=Inherit: Same as input
  b(352) : Gain  Gain=0.00230359584321299495  ParamDataTypeStr=double  RndMeth=Nearest  SaturateOnIntegerOverflow=on  OutDataTypeStr=Inherit: Same as input
  b(353) : Gain  Gain=0.00261576565085099412  ParamDataTypeStr=double  RndMeth=Nearest  SaturateOnIntegerOverflow=on  OutDataTypeStr=Inherit: Same as input
  b(354) : Gain  Gain=0.00290736343473789721  ParamDataTypeStr=double  RndMeth=Nearest  SaturateOnIntegerOverflow=on  OutDataTypeStr=Inherit: Same as input
  b(355) : Gain  Gain=0.00317830525562316476  ParamDataTypeStr=double  RndMeth=Nearest  SaturateOnIntegerOverflow=on  OutDataTypeStr=Inherit: Same as input
  b(356) : Gain  Gain=0.00342754062478000223  ParamDataTypeStr=double  RndMeth=Nearest  SaturateOnIntegerOverflow=on  OutDataTypeStr=Inherit: Same as input
  b(357) : Gain  Gain=0.00365524307304546667  ParamDataTypeStr=double  RndMeth=Nearest  SaturateOnIntegerOverflow=on  OutDataTypeStr=Inherit: Same as input
  b(358) : Gain  Gain=0.00386057987620588502  ParamDataTypeStr=double  RndMeth=Nearest  SaturateOnIntegerOverflow=on  OutDataTypeStr=Inherit: Same as input
  b(359) : Gain  Gain=0.00404392562049606889  ParamDataTypeStr=double  RndMeth=Nearest  SaturateOnIntegerOverflow=on  OutDataTypeStr=Inherit: Same as input
  b(36) : Gain  Gain=-0.000244422722580023592  ParamDataTypeStr=double  RndMeth=Nearest  SaturateOnIntegerOverflow=on  OutDataTypeStr=Inherit: Same as input
  b(360) : Gain  Gain=0.00420466577279327014  ParamDataTypeStr=double  RndMeth=Nearest  SaturateOnIntegerOverflow=on  OutDataTypeStr=Inherit: Same as input
  b(361) : Gain  Gain=0.00434340083942166052  ParamDataTypeStr=double  RndMeth=Nearest  SaturateOnIntegerOverflow=on  OutDataTypeStr=Inherit: Same as input
  b(362) : Gain  Gain=0.00445973230065942021  ParamDataTypeStr=double  RndMeth=Nearest  SaturateOnIntegerOverflow=on  OutDataTypeStr=Inherit: Same as input
  b(363) : Gain  Gain=0.00455448397919440591  ParamDataTypeStr=double  RndMeth=Nearest  SaturateOnIntegerOverflow=on  OutDataTypeStr=Inherit: Same as input
  b(364) : Gain  Gain=0.00462737166796193655  ParamDataTypeStr=double  RndMeth=Nearest  SaturateOnIntegerOverflow=on  OutDataTypeStr=Inherit: Same as input
  b(365) : Gain  Gain=0.00467948532462431933  ParamDataTypeStr=double  RndMeth=Nearest  SaturateOnIntegerOverflow=on  OutDataTypeStr=Inherit: Same as input
  b(366) : Gain  Gain=0.00471069265375758696  ParamDataTypeStr=double  RndMeth=Nearest  SaturateOnIntegerOverflow=on  OutDataTypeStr=Inherit: Same as input
  b(367) : Gain  Gain=0.00472223215326236789  ParamDataTypeStr=double  RndMeth=Nearest  SaturateOnIntegerOverflow=on  OutDataTypeStr=Inherit: Same as input
  b(368) : Gain  Gain=0.00471414582817185693  ParamDataTypeStr=double  RndMeth=Nearest  SaturateOnIntegerOverflow=on  OutDataTypeStr=Inherit: Same as input
  b(369) : Gain  Gain=0.00468784260596036978  ParamDataTypeStr=double  RndMeth=Nearest  SaturateOnIntegerOverflow=on  OutDataTypeStr=Inherit: Same as input
  b(37) : Gain  Gain=-0.000263040701395831364  ParamDataTypeStr=double  RndMeth=Nearest  SaturateOnIntegerOverflow=on  OutDataTypeStr=Inherit: Same as input
  b(370) : Gain  Gain=0.00464346418155206584  ParamDataTypeStr=double  RndMeth=Nearest  SaturateOnIntegerOverflow=on  OutDataTypeStr=Inherit: Same as input
  b(371) : Gain  Gain=0.00458254074599091094  ParamDataTypeStr=double  RndMeth=Nearest  SaturateOnIntegerOverflow=on  OutDataTypeStr=Inherit: Same as input
  b(372) : Gain  Gain=0.00450533688353090857  ParamDataTypeStr=double  RndMeth=Nearest  SaturateOnIntegerOverflow=on  OutDataTypeStr=Inherit: Same as input
  b(373) : Gain  Gain=0.00441351242527037672  ParamDataTypeStr=double  RndMeth=Nearest  SaturateOnIntegerOverflow=on  OutDataTypeStr=Inherit: Same as input
  b(374) : Gain  Gain=0.0043073826617828579  ParamDataTypeStr=double  RndMeth=Nearest  SaturateOnIntegerOverflow=on  OutDataTypeStr=Inherit: Same as input
  b(375) : Gain  Gain=0.00418867978645957092  ParamDataTypeStr=double  RndMeth=Nearest  SaturateOnIntegerOverflow=on  OutDataTypeStr=Inherit: Same as input
  b(376) : Gain  Gain=0.00405777405273261005  ParamDataTypeStr=double  RndMeth=Nearest  SaturateOnIntegerOverflow=on  OutDataTypeStr=Inherit: Same as input
  b(377) : Gain  Gain=0.00391645258241414898  ParamDataTypeStr=double  RndMeth=Nearest  SaturateOnIntegerOverflow=on  OutDataTypeStr=Inherit: Same as input
  b(378) : Gain  Gain=0.00376516794268936172  ParamDataTypeStr=double  RndMeth=Nearest  SaturateOnIntegerOverflow=on  OutDataTypeStr=Inherit: Same as input
  b(379) : Gain  Gain=0.00360564932851902388  ParamDataTypeStr=double  RndMeth=Nearest  SaturateOnIntegerOverflow=on  OutDataTypeStr=Inherit: Same as input
  b(38) : Gain  Gain=-0.000280358987114503935  ParamDataTypeStr=double  RndMeth=Nearest  SaturateOnIntegerOverflow=on  OutDataTypeStr=Inherit: Same as input
  b(380) : Gain  Gain=0.00343839387437318202  ParamDataTypeStr=double  RndMeth=Nearest  SaturateOnIntegerOverflow=on  OutDataTypeStr=Inherit: Same as input
  b(381) : Gain  Gain=0.00326516612697404403  ParamDataTypeStr=double  RndMeth=Nearest  SaturateOnIntegerOverflow=on  OutDataTypeStr=Inherit: Same as input
  b(382) : Gain  Gain=0.00308638207372412135  ParamDataTypeStr=double  RndMeth=Nearest  SaturateOnIntegerOverflow=on  OutDataTypeStr=Inherit: Same as input
  b(383) : Gain  Gain=0.00290381159203095124  ParamDataTypeStr=double  RndMeth=Nearest  SaturateOnIntegerOverflow=on  OutDataTypeStr=Inherit: Same as input
  b(384) : Gain  Gain=0.0027178557454954292  ParamDataTypeStr=double  RndMeth=Nearest  SaturateOnIntegerOverflow=on  OutDataTypeStr=Inherit: Same as input
  b(385) : Gain  Gain=0.00253023101632903575  ParamDataTypeStr=double  RndMeth=Nearest  SaturateOnIntegerOverflow=on  OutDataTypeStr=Inherit: Same as input
  b(386) : Gain  Gain=0.00234124102603082635  ParamDataTypeStr=double  RndMeth=Nearest  SaturateOnIntegerOverflow=on  OutDataTypeStr=Inherit: Same as input
  b(387) : Gain  Gain=0.00215255509300310262  ParamDataTypeStr=double  RndMeth=Nearest  SaturateOnIntegerOverflow=on  OutDataTypeStr=Inherit: Same as input
  b(388) : Gain  Gain=0.0019644273961855049  ParamDataTypeStr=double  RndMeth=Nearest  SaturateOnIntegerOverflow=on  OutDataTypeStr=Inherit: Same as input
  b(389) : Gain  Gain=0.00177845198936645564  ParamDataTypeStr=double  RndMeth=Nearest  SaturateOnIntegerOverflow=on  OutDataTypeStr=Inherit: Same as input
  b(39) : Gain  Gain=-0.000297528049151355107  ParamDataTypeStr=double  RndMeth=Nearest  SaturateOnIntegerOverflow=on  OutDataTypeStr=Inherit: Same as input
  b(390) : Gain  Gain=0.00159476176493942136  ParamDataTypeStr=double  RndMeth=Nearest  SaturateOnIntegerOverflow=on  OutDataTypeStr=Inherit: Same as input
  b(391) : Gain  Gain=0.00141487218687043554  ParamDataTypeStr=double  RndMeth=Nearest  SaturateOnIntegerOverflow=on  OutDataTypeStr=Inherit: Same as input
  b(392) : Gain  Gain=0.00123877378306479539  ParamDataTypeStr=double  RndMeth=Nearest  SaturateOnIntegerOverflow=on  OutDataTypeStr=Inherit: Same as input
  b(393) : Gain  Gain=0.00106797088471714927  ParamDataTypeStr=double  RndMeth=Nearest  SaturateOnIntegerOverflow=on  OutDataTypeStr=Inherit: Same as input
  b(394) : Gain  Gain=0.000902265678969772192  ParamDataTypeStr=double  RndMeth=Nearest  SaturateOnIntegerOverflow=on  OutDataTypeStr=Inherit: Same as input
  b(395) : Gain  Gain=0.000743040070891614452  ParamDataTypeStr=double  RndMeth=Nearest  SaturateOnIntegerOverflow=on  OutDataTypeStr=Inherit: Same as input
  b(396) : Gain  Gain=0.000590057589736560101  ParamDataTypeStr=double  RndMeth=Nearest  SaturateOnIntegerOverflow=on  OutDataTypeStr=Inherit: Same as input
  b(397) : Gain  Gain=0.000444512367971374497  ParamDataTypeStr=double  RndMeth=Nearest  SaturateOnIntegerOverflow=on  OutDataTypeStr=Inherit: Same as input
  b(398) : Gain  Gain=0.000306041227612374213  ParamDataTypeStr=double  RndMeth=Nearest  SaturateOnIntegerOverflow=on  OutDataTypeStr=Inherit: Same as input
  b(399) : Gain  Gain=0.000175769318122429323  ParamDataTypeStr=double  RndMeth=Nearest  SaturateOnIntegerOverflow=on  OutDataTypeStr=Inherit: Same as input
  b(4) : Gain  Gain=0.000126958318748944705  ParamDataTypeStr=double  RndMeth=Nearest  SaturateOnIntegerOverflow=on  OutDataTypeStr=Inherit: Same as input
  b(40) : Gain  Gain=-0.000313246594477974757  ParamDataTypeStr=double  RndMeth=Nearest  SaturateOnIntegerOverflow=on  OutDataTypeStr=Inherit: Same as input
  b(400) : Gain  Gain=5.3221221105915692e-05  ParamDataTypeStr=double  RndMeth=Nearest  SaturateOnIntegerOverflow=on  OutDataTypeStr=Inherit: Same as input
  b(401) : Gain  Gain=-6.06350808818785243e-05  ParamDataTypeStr=double  RndMeth=Nearest  SaturateOnIntegerOverflow=on  OutDataTypeStr=Inherit: Same as input
  b(402) : Gain  Gain=-0.000166409873705706049  ParamDataTypeStr=double  RndMeth=Nearest  SaturateOnIntegerOverflow=on  OutDataTypeStr=Inherit: Same as input
  b(403) : Gain  Gain=-0.000263221131644026524  ParamDataTypeStr=double  RndMeth=Nearest  SaturateOnIntegerOverflow=on  OutDataTypeStr=Inherit: Same as input
  b(404) : Gain  Gain=-0.000351769691493805832  ParamDataTypeStr=double  RndMeth=Nearest  SaturateOnIntegerOverflow=on  OutDataTypeStr=Inherit: Same as input
  b(405) : Gain  Gain=-0.000431307266994649828  ParamDataTypeStr=double  RndMeth=Nearest  SaturateOnIntegerOverflow=on  OutDataTypeStr=Inherit: Same as input
  b(406) : Gain  Gain=-0.000502625089221949307  ParamDataTypeStr=double  RndMeth=Nearest  SaturateOnIntegerOverflow=on  OutDataTypeStr=Inherit: Same as input
  b(407) : Gain  Gain=-0.000565134472783350244  ParamDataTypeStr=double  RndMeth=Nearest  SaturateOnIntegerOverflow=on  OutDataTypeStr=Inherit: Same as input
  b(408) : Gain  Gain=-0.000619640367190464419  ParamDataTypeStr=double  RndMeth=Nearest  SaturateOnIntegerOverflow=on  OutDataTypeStr=Inherit: Same as input
  b(409) : Gain  Gain=-0.000665646484304962876  ParamDataTypeStr=double  RndMeth=Nearest  SaturateOnIntegerOverflow=on  OutDataTypeStr=Inherit: Same as input
  b(41) : Gain  Gain=-0.000328550564974419397  ParamDataTypeStr=double  RndMeth=Nearest  SaturateOnIntegerOverflow=on  OutDataTypeStr=Inherit: Same as input
  b(410) : Gain  Gain=-0.000704141633403310195  ParamDataTypeStr=double  RndMeth=Nearest  SaturateOnIntegerOverflow=on  OutDataTypeStr=Inherit: Same as input
  b(411) : Gain  Gain=-0.000734569828311722726  ParamDataTypeStr=double  RndMeth=Nearest  SaturateOnIntegerOverflow=on  OutDataTypeStr=Inherit: Same as input
  b(412) : Gain  Gain=-0.00075805870009854092  ParamDataTypeStr=double  RndMeth=Nearest  SaturateOnIntegerOverflow=on  OutDataTypeStr=Inherit: Same as input
  b(413) : Gain  Gain=-0.000774164375811770954  ParamDataTypeStr=double  RndMeth=Nearest  SaturateOnIntegerOverflow=on  OutDataTypeStr=Inherit: Same as input
  b(414) : Gain  Gain=-0.00078403753021555095  ParamDataTypeStr=double  RndMeth=Nearest  SaturateOnIntegerOverflow=on  OutDataTypeStr=Inherit: Same as input
  b(415) : Gain  Gain=-0.000787233425354552717  ParamDataTypeStr=double  RndMeth=Nearest  SaturateOnIntegerOverflow=on  OutDataTypeStr=Inherit: Same as input
  b(416) : Gain  Gain=-0.000784985189046555625  ParamDataTypeStr=double  RndMeth=Nearest  SaturateOnIntegerOverflow=on  OutDataTypeStr=Inherit: Same as input
  b(417) : Gain  Gain=-0.000776912328953108179  ParamDataTypeStr=double  RndMeth=Nearest  SaturateOnIntegerOverflow=on  OutDataTypeStr=Inherit: Same as input
  b(418) : Gain  Gain=-0.000764284945513389754  ParamDataTypeStr=double  RndMeth=Nearest  SaturateOnIntegerOverflow=on  OutDataTypeStr=Inherit: Same as input
  b(419) : Gain  Gain=-0.000746694212294661563  ParamDataTypeStr=double  RndMeth=Nearest  SaturateOnIntegerOverflow=on  OutDataTypeStr=Inherit: Same as input
  b(42) : Gain  Gain=-0.000342087513098722614  ParamDataTypeStr=double  RndMeth=Nearest  SaturateOnIntegerOverflow=on  OutDataTypeStr=Inherit: Same as input
  b(420) : Gain  Gain=-0.000725457005707568739  ParamDataTypeStr=double  RndMeth=Nearest  SaturateOnIntegerOverflow=on  OutDataTypeStr=Inherit: Same as input
  b(421) : Gain  Gain=-0.000700138237773947664  ParamDataTypeStr=double  RndMeth=Nearest  SaturateOnIntegerOverflow=on  OutDataTypeStr=Inherit: Same as input
  b(422) : Gain  Gain=-0.000672143479130331268  ParamDataTypeStr=double  RndMeth=Nearest  SaturateOnIntegerOverflow=on  OutDataTypeStr=Inherit: Same as input
  b(423) : Gain  Gain=-0.000640997939764448256  ParamDataTypeStr=double  RndMeth=Nearest  SaturateOnIntegerOverflow=on  OutDataTypeStr=Inherit: Same as input
  b(424) : Gain  Gain=-0.000608018296520356112  ParamDataTypeStr=double  RndMeth=Nearest  SaturateOnIntegerOverflow=on  OutDataTypeStr=Inherit: Same as input
  b(425) : Gain  Gain=-0.00057288638177031251  ParamDataTypeStr=double  RndMeth=Nearest  SaturateOnIntegerOverflow=on  OutDataTypeStr=Inherit: Same as input
  b(426) : Gain  Gain=-0.000536759002049947602  ParamDataTypeStr=double  RndMeth=Nearest  SaturateOnIntegerOverflow=on  OutDataTypeStr=Inherit: Same as input
  b(427) : Gain  Gain=-0.000499272274876905349  ParamDataTypeStr=double  RndMeth=Nearest  SaturateOnIntegerOverflow=on  OutDataTypeStr=Inherit: Same as input
  b(428) : Gain  Gain=-0.000461669334225578475  ParamDataTypeStr=double  RndMeth=Nearest  SaturateOnIntegerOverflow=on  OutDataTypeStr=Inherit: Same as input
  b(429) : Gain  Gain=-0.000423533495409219316  ParamDataTypeStr=double  RndMeth=Nearest  SaturateOnIntegerOverflow=on  OutDataTypeStr=Inherit: Same as input
  b(43) : Gain  Gain=-0.000354911467429252061  ParamDataTypeStr=double  RndMeth=Nearest  SaturateOnIntegerOverflow=on  OutDataTypeStr=Inherit: Same as input
  b(430) : Gain  Gain=-0.000386007594417995138  ParamDataTypeStr=double  RndMeth=Nearest  SaturateOnIntegerOverflow=on  OutDataTypeStr=Inherit: Same as input
  b(431) : Gain  Gain=-0.000348624240333695939  ParamDataTypeStr=double  RndMeth=Nearest  SaturateOnIntegerOverflow=on  OutDataTypeStr=Inherit: Same as input
  b(432) : Gain  Gain=-0.000312529436229563081  ParamDataTypeStr=double  RndMeth=Nearest  SaturateOnIntegerOverflow=on  OutDataTypeStr=Inherit: Same as input
  b(433) : Gain  Gain=-0.00027723555258353798  ParamDataTypeStr=double  RndMeth=Nearest  SaturateOnIntegerOverflow=on  OutDataTypeStr=Inherit: Same as input
  b(434) : Gain  Gain=-0.000243803841427045562  ParamDataTypeStr=double  RndMeth=Nearest  SaturateOnIntegerOverflow=on  OutDataTypeStr=Inherit: Same as input
  b(435) : Gain  Gain=-0.000211695078287365548  ParamDataTypeStr=double  RndMeth=Nearest  SaturateOnIntegerOverflow=on  OutDataTypeStr=Inherit: Same as input
  b(436) : Gain  Gain=-0.00018187967171705505  ParamDataTypeStr=double  RndMeth=Nearest  SaturateOnIntegerOverflow=on  OutDataTypeStr=Inherit: Same as input
  b(437) : Gain  Gain=-0.000153800533059332729  ParamDataTypeStr=double  RndMeth=Nearest  SaturateOnIntegerOverflow=on  OutDataTypeStr=Inherit: Same as input
  b(438) : Gain  Gain=-0.00012844573614923015  ParamDataTypeStr=double  RndMeth=Nearest  SaturateOnIntegerOverflow=on  OutDataTypeStr=Inherit: Same as input
  b(439) : Gain  Gain=-0.000104999200466021321  ParamDataTypeStr=double  RndMeth=Nearest  SaturateOnIntegerOverflow=on  OutDataTypeStr=Inherit: Same as input
  b(44) : Gain  Gain=-0.000365845398302402621  ParamDataTypeStr=double  RndMeth=Nearest  SaturateOnIntegerOverflow=on  OutDataTypeStr=Inherit: Same as input
  b(440) : Gain  Gain=-8.46336706624266095e-05  ParamDataTypeStr=double  RndMeth=Nearest  SaturateOnIntegerOverflow=on  OutDataTypeStr=Inherit: Same as input
  b(441) : Gain  Gain=-6.63999170443811595e-05  ParamDataTypeStr=double  RndMeth=Nearest  SaturateOnIntegerOverflow=on  OutDataTypeStr=Inherit: Same as input
  b(442) : Gain  Gain=-5.127065973762235e-05  ParamDataTypeStr=double  RndMeth=Nearest  SaturateOnIntegerOverflow=on  OutDataTypeStr=Inherit: Same as input
  b(443) : Gain  Gain=-3.83862678230118774e-05  ParamDataTypeStr=double  RndMeth=Nearest  SaturateOnIntegerOverflow=on  OutDataTypeStr=Inherit: Same as input
  b(444) : Gain  Gain=-2.87166278037361087e-05  ParamDataTypeStr=double  RndMeth=Nearest  SaturateOnIntegerOverflow=on  OutDataTypeStr=Inherit: Same as input
  b(445) : Gain  Gain=-2.12850613980476808e-05  ParamDataTypeStr=double  RndMeth=Nearest  SaturateOnIntegerOverflow=on  OutDataTypeStr=Inherit: Same as input
  b(446) : Gain  Gain=-1.69628308546508448e-05  ParamDataTypeStr=double  RndMeth=Nearest  SaturateOnIntegerOverflow=on  OutDataTypeStr=Inherit: Same as input
  b(447) : Gain  Gain=-1.47437363230819383e-05  ParamDataTypeStr=double  RndMeth=Nearest  SaturateOnIntegerOverflow=on  OutDataTypeStr=Inherit: Same as input
  b(448) : Gain  Gain=-1.55128158049954671e-05  ParamDataTypeStr=double  RndMeth=Nearest  SaturateOnIntegerOverflow=on  OutDataTypeStr=Inherit: Same as input
  b(449) : Gain  Gain=-1.82129216426999644e-05  ParamDataTypeStr=double  RndMeth=Nearest  SaturateOnIntegerOverflow=on  OutDataTypeStr=Inherit: Same as input
  b(45) : Gain  Gain=-0.000376157350598188729  ParamDataTypeStr=double  RndMeth=Nearest  SaturateOnIntegerOverflow=on  OutDataTypeStr=Inherit: Same as input
  b(450) : Gain  Gain=-2.36957211731823793e-05  ParamDataTypeStr=double  RndMeth=Nearest  SaturateOnIntegerOverflow=on  OutDataTypeStr=Inherit: Same as input
  b(451) : Gain  Gain=-3.08383793457291371e-05  ParamDataTypeStr=double  RndMeth=Nearest  SaturateOnIntegerOverflow=on  OutDataTypeStr=Inherit: Same as input
  b(452) : Gain  Gain=-4.04269010002347978e-05  ParamDataTypeStr=double  RndMeth=Nearest  SaturateOnIntegerOverflow=on  OutDataTypeStr=Inherit: Same as input
  b(453) : Gain  Gain=-5.15015329802558704e-05  ParamDataTypeStr=double  RndMeth=Nearest  SaturateOnIntegerOverflow=on  OutDataTypeStr=Inherit: Same as input
  b(454) : Gain  Gain=-6.45312083203074521e-05  ParamDataTypeStr=double  RndMeth=Nearest  SaturateOnIntegerOverflow=on  OutDataTypeStr=Inherit: Same as input
  b(455) : Gain  Gain=-7.87286212535760581e-05  ParamDataTypeStr=double  RndMeth=Nearest  SaturateOnIntegerOverflow=on  OutDataTypeStr=Inherit: Same as input
  b(456) : Gain  Gain=-9.46829036739340896e-05  ParamDataTypeStr=double  RndMeth=Nearest  SaturateOnIntegerOverflow=on  OutDataTypeStr=Inherit: Same as input
  b(457) : Gain  Gain=-0.00011125252133578384  ParamDataTypeStr=double  RndMeth=Nearest  SaturateOnIntegerOverflow=on  OutDataTypeStr=Inherit: Same as input
  b(458) : Gain  Gain=-0.000129141873349178935  ParamDataTypeStr=double  RndMeth=Nearest  SaturateOnIntegerOverflow=on  OutDataTypeStr=Inherit: Same as input
  b(459) : Gain  Gain=-0.000147315132967771201  ParamDataTypeStr=double  RndMeth=Nearest  SaturateOnIntegerOverflow=on  OutDataTypeStr=Inherit: Same as input
  b(46) : Gain  Gain=-0.000384291427222763172  ParamDataTypeStr=double  RndMeth=Nearest  SaturateOnIntegerOverflow=on  OutDataTypeStr=Inherit: Same as input
  b(460) : Gain  Gain=-0.000166478229983800735  ParamDataTypeStr=double  RndMeth=Nearest  SaturateOnIntegerOverflow=on  OutDataTypeStr=Inherit: Same as input
  b(461) : Gain  Gain=-0.000185503270808741157  ParamDataTypeStr=double  RndMeth=Nearest  SaturateOnIntegerOverflow=on  OutDataTypeStr=Inherit: Same as input
  b(462) : Gain  Gain=-0.00020509011935799723  ParamDataTypeStr=double  RndMeth=Nearest  SaturateOnIntegerOverflow=on  OutDataTypeStr=Inherit: Same as input
  b(463) : Gain  Gain=-0.00022414279328602355  ParamDataTypeStr=double  RndMeth=Nearest  SaturateOnIntegerOverflow=on  OutDataTypeStr=Inherit: Same as input
  b(464) : Gain  Gain=-0.000243411438438570623  ParamDataTypeStr=double  RndMeth=Nearest  SaturateOnIntegerOverflow=on  OutDataTypeStr=Inherit: Same as input
  b(465) : Gain  Gain=-0.000261789142866730284  ParamDataTypeStr=double  RndMeth=Nearest  SaturateOnIntegerOverflow=on  OutDataTypeStr=Inherit: Same as input
  b(466) : Gain  Gain=-0.000280071574432796044  ParamDataTypeStr=double  RndMeth=Nearest  SaturateOnIntegerOverflow=on  OutDataTypeStr=Inherit: Same as input
  b(467) : Gain  Gain=-0.000296990192063201945  ParamDataTypeStr=double  RndMeth=Nearest  SaturateOnIntegerOverflow=on  OutDataTypeStr=Inherit: Same as input
  b(468) : Gain  Gain=-0.000313697423958395668  ParamDataTypeStr=double  RndMeth=Nearest  SaturateOnIntegerOverflow=on  OutDataTypeStr=Inherit: Same as input
  b(469) : Gain  Gain=-0.000328612037461096336  ParamDataTypeStr=double  RndMeth=Nearest  SaturateOnIntegerOverflow=on  OutDataTypeStr=Inherit: Same as input
  b(47) : Gain  Gain=-0.000391134875770449662  ParamDataTypeStr=double  RndMeth=Nearest  SaturateOnIntegerOverflow=on  OutDataTypeStr=Inherit: Same as input
  b(470) : Gain  Gain=-0.000342894954706609613  ParamDataTypeStr=double  RndMeth=Nearest  SaturateOnIntegerOverflow=on  OutDataTypeStr=Inherit: Same as input
  b(471) : Gain  Gain=-0.000355511706333689866  ParamDataTypeStr=double  RndMeth=Nearest  SaturateOnIntegerOverflow=on  OutDataTypeStr=Inherit: Same as input
  b(472) : Gain  Gain=-0.000367171401728139373  ParamDataTypeStr=double  RndMeth=Nearest  SaturateOnIntegerOverflow=on  OutDataTypeStr=Inherit: Same as input
  b(473) : Gain  Gain=-0.000376818546642253716  ParamDataTypeStr=double  RndMeth=Nearest  SaturateOnIntegerOverflow=on  OutDataTypeStr=Inherit: Same as input
  b(474) : Gain  Gain=-0.000385359957846202793  ParamDataTypeStr=double  RndMeth=Nearest  SaturateOnIntegerOverflow=on  OutDataTypeStr=Inherit: Same as input
  b(475) : Gain  Gain=-0.000391841892495430836  ParamDataTypeStr=double  RndMeth=Nearest  SaturateOnIntegerOverflow=on  OutDataTypeStr=Inherit: Same as input
  b(476) : Gain  Gain=-0.000397125758577358606  ParamDataTypeStr=double  RndMeth=Nearest  SaturateOnIntegerOverflow=on  OutDataTypeStr=Inherit: Same as input
  b(477) : Gain  Gain=-0.00040023311630166215  ParamDataTypeStr=double  RndMeth=Nearest  SaturateOnIntegerOverflow=on  OutDataTypeStr=Inherit: Same as input
  b(478) : Gain  Gain=-0.000402035792474276111  ParamDataTypeStr=double  RndMeth=Nearest  SaturateOnIntegerOverflow=on  OutDataTypeStr=Inherit: Same as input
  b(479) : Gain  Gain=-0.000401659938941869958  ParamDataTypeStr=double  RndMeth=Nearest  SaturateOnIntegerOverflow=on  OutDataTypeStr=Inherit: Same as input
  b(48) : Gain  Gain=-0.000396279890881591403  ParamDataTypeStr=double  RndMeth=Nearest  SaturateOnIntegerOverflow=on  OutDataTypeStr=Inherit: Same as input
  b(480) : Gain  Gain=-0.000399976844345353204  ParamDataTypeStr=double  RndMeth=Nearest  SaturateOnIntegerOverflow=on  OutDataTypeStr=Inherit: Same as input
  b(481) : Gain  Gain=-0.000396279890881591403  ParamDataTypeStr=double  RndMeth=Nearest  SaturateOnIntegerOverflow=on  OutDataTypeStr=Inherit: Same as input
  b(482) : Gain  Gain=-0.000391134875770449662  ParamDataTypeStr=double  RndMeth=Nearest  SaturateOnIntegerOverflow=on  OutDataTypeStr=Inherit: Same as input
  b(483) : Gain  Gain=-0.000384291427222763172  ParamDataTypeStr=double  RndMeth=Nearest  SaturateOnIntegerOverflow=on  OutDataTypeStr=Inherit: Same as input
  b(484) : Gain  Gain=-0.000376157350598188729  ParamDataTypeStr=double  RndMeth=Nearest  SaturateOnIntegerOverflow=on  OutDataTypeStr=Inherit: Same as input
  b(485) : Gain  Gain=-0.000365845398302402621  ParamDataTypeStr=double  RndMeth=Nearest  SaturateOnIntegerOverflow=on  OutDataTypeStr=Inherit: Same as input
  b(486) : Gain  Gain=-0.000354911467429252061  ParamDataTypeStr=double  RndMeth=Nearest  SaturateOnIntegerOverflow=on  OutDataTypeStr=Inherit: Same as input
  b(487) : Gain  Gain=-0.000342087513098722614  ParamDataTypeStr=double  RndMeth=Nearest  SaturateOnIntegerOverflow=on  OutDataTypeStr=Inherit: Same as input
  b(488) : Gain  Gain=-0.000328550564974419397  ParamDataTypeStr=double  RndMeth=Nearest  SaturateOnIntegerOverflow=on  OutDataTypeStr=Inherit: Same as input
  b(489) : Gain  Gain=-0.000313246594477974757  ParamDataTypeStr=double  RndMeth=Nearest  SaturateOnIntegerOverflow=on  OutDataTypeStr=Inherit: Same as input
  b(49) : Gain  Gain=-0.000399976844345353204  ParamDataTypeStr=double  RndMeth=Nearest  SaturateOnIntegerOverflow=on  OutDataTypeStr=Inherit: Same as input
  b(490) : Gain  Gain=-0.000297528049151355107  ParamDataTypeStr=double  RndMeth=Nearest  SaturateOnIntegerOverflow=on  OutDataTypeStr=Inherit: Same as input
  b(491) : Gain  Gain=-0.000280358987114503935  ParamDataTypeStr=double  RndMeth=Nearest  SaturateOnIntegerOverflow=on  OutDataTypeStr=Inherit: Same as input
  b(492) : Gain  Gain=-0.000263040701395831364  ParamDataTypeStr=double  RndMeth=Nearest  SaturateOnIntegerOverflow=on  OutDataTypeStr=Inherit: Same as input
  b(493) : Gain  Gain=-0.000244422722580023592  ParamDataTypeStr=double  RndMeth=Nearest  SaturateOnIntegerOverflow=on  OutDataTypeStr=Inherit: Same as input
  b(494) : Gain  Gain=-0.000225875280666558518  ParamDataTypeStr=double  RndMeth=Nearest  SaturateOnIntegerOverflow=on  OutDataTypeStr=Inherit: Same as input
  b(495) : Gain  Gain=-0.000206139072550225958  ParamDataTypeStr=double  RndMeth=Nearest  SaturateOnIntegerOverflow=on  OutDataTypeStr=Inherit: Same as input
  b(496) : Gain  Gain=-0.000186903105556324297  ParamDataTypeStr=double  RndMeth=Nearest  SaturateOnIntegerOverflow=on  OutDataTypeStr=Inherit: Same as input
  b(497) : Gain  Gain=-0.000166417949659631399  ParamDataTypeStr=double  RndMeth=Nearest  SaturateOnIntegerOverflow=on  OutDataTypeStr=Inherit: Same as input
  b(498) : Gain  Gain=-0.000146832212862152119  ParamDataTypeStr=double  RndMeth=Nearest  SaturateOnIntegerOverflow=on  OutDataTypeStr=Inherit: Same as input
  b(499) : Gain  Gain=-0.000127069818868432967  ParamDataTypeStr=double  RndMeth=Nearest  SaturateOnIntegerOverflow=on  OutDataTypeStr=Inherit: Same as input
  b(5) : Gain  Gain=0.000129014399545789677  ParamDataTypeStr=double  RndMeth=Nearest  SaturateOnIntegerOverflow=on  OutDataTypeStr=Inherit: Same as input
  b(50) : Gain  Gain=-0.000401659938941869958  ParamDataTypeStr=double  RndMeth=Nearest  SaturateOnIntegerOverflow=on  OutDataTypeStr=Inherit: Same as input
  b(500) : Gain  Gain=-0.000106978433770536828  ParamDataTypeStr=double  RndMeth=Nearest  SaturateOnIntegerOverflow=on  OutDataTypeStr=Inherit: Same as input
  b(501) : Gain  Gain=-8.73504816807577078e-05  ParamDataTypeStr=double  RndMeth=Nearest  SaturateOnIntegerOverflow=on  OutDataTypeStr=Inherit: Same as input
  b(502) : Gain  Gain=-6.84426124636459271e-05  ParamDataTypeStr=double  RndMeth=Nearest  SaturateOnIntegerOverflow=on  OutDataTypeStr=Inherit: Same as input
  b(503) : Gain  Gain=-4.98086298525179418e-05  ParamDataTypeStr=double  RndMeth=Nearest  SaturateOnIntegerOverflow=on  OutDataTypeStr=Inherit: Same as input
  b(504) : Gain  Gain=-3.18260172032644104e-05  ParamDataTypeStr=double  RndMeth=Nearest  SaturateOnIntegerOverflow=on  OutDataTypeStr=Inherit: Same as input
  b(505) : Gain  Gain=-1.41991623558972851e-05  ParamDataTypeStr=double  RndMeth=Nearest  SaturateOnIntegerOverflow=on  OutDataTypeStr=Inherit: Same as input
  b(506) : Gain  Gain=2.53229324894679517e-06  ParamDataTypeStr=double  RndMeth=Nearest  SaturateOnIntegerOverflow=on  OutDataTypeStr=Inherit: Same as input
  b(507) : Gain  Gain=1.85707383679374095e-05  ParamDataTypeStr=double  RndMeth=Nearest  SaturateOnIntegerOverflow=on  OutDataTypeStr=Inherit: Same as input
  b(508) : Gain  Gain=3.35500754738617818e-05  ParamDataTypeStr=double  RndMeth=Nearest  SaturateOnIntegerOverflow=on  OutDataTypeStr=Inherit: Same as input
  b(509) : Gain  Gain=4.75559208421214279e-05  ParamDataTypeStr=double  RndMeth=Nearest  SaturateOnIntegerOverflow=on  OutDataTypeStr=Inherit: Same as input
  b(51) : Gain  Gain=-0.000402035792474276111  ParamDataTypeStr=double  RndMeth=Nearest  SaturateOnIntegerOverflow=on  OutDataTypeStr=Inherit: Same as input
  b(510) : Gain  Gain=6.06151093979667883e-05  ParamDataTypeStr=double  RndMeth=Nearest  SaturateOnIntegerOverflow=on  OutDataTypeStr=Inherit: Same as input
  b(511) : Gain  Gain=7.22562062001517146e-05  ParamDataTypeStr=double  RndMeth=Nearest  SaturateOnIntegerOverflow=on  OutDataTypeStr=Inherit: Same as input
  b(512) : Gain  Gain=8.34713962025901597e-05  ParamDataTypeStr=double  RndMeth=Nearest  SaturateOnIntegerOverflow=on  OutDataTypeStr=Inherit: Same as input
  b(513) : Gain  Gain=9.42827838523885992e-05  ParamDataTypeStr=double  RndMeth=Nearest  SaturateOnIntegerOverflow=on  OutDataTypeStr=Inherit: Same as input
  b(514) : Gain  Gain=0.000100118512988072762  ParamDataTypeStr=double  RndMeth=Nearest  SaturateOnIntegerOverflow=on  OutDataTypeStr=Inherit: Same as input
  b(515) : Gain  Gain=0.000109424395758821007  ParamDataTypeStr=double  RndMeth=Nearest  SaturateOnIntegerOverflow=on  OutDataTypeStr=Inherit: Same as input
  b(516) : Gain  Gain=0.000115908705622264248  ParamDataTypeStr=double  RndMeth=Nearest  SaturateOnIntegerOverflow=on  OutDataTypeStr=Inherit: Same as input
  b(517) : Gain  Gain=0.000122046249196258033  ParamDataTypeStr=double  RndMeth=Nearest  SaturateOnIntegerOverflow=on  OutDataTypeStr=Inherit: Same as input
  b(518) : Gain  Gain=0.000125642526667612978  ParamDataTypeStr=double  RndMeth=Nearest  SaturateOnIntegerOverflow=on  OutDataTypeStr=Inherit: Same as input
  b(519) : Gain  Gain=0.000128994813916388394  ParamDataTypeStr=double  RndMeth=Nearest  SaturateOnIntegerOverflow=on  OutDataTypeStr=Inherit: Same as input
  b(52) : Gain  Gain=-0.00040023311630166215  ParamDataTypeStr=double  RndMeth=Nearest  SaturateOnIntegerOverflow=on  OutDataTypeStr=Inherit: Same as input
  b(520) : Gain  Gain=0.000130387945813979691  ParamDataTypeStr=double  RndMeth=Nearest  SaturateOnIntegerOverflow=on  OutDataTypeStr=Inherit: Same as input
  b(521) : Gain  Gain=0.000131740041189622225  ParamDataTypeStr=double  RndMeth=Nearest  SaturateOnIntegerOverflow=on  OutDataTypeStr=Inherit: Same as input
  b(522) : Gain  Gain=0.000131388393933855882  ParamDataTypeStr=double  RndMeth=Nearest  SaturateOnIntegerOverflow=on  OutDataTypeStr=Inherit: Same as input
  b(523) : Gain  Gain=0.000131022132570349182  ParamDataTypeStr=double  RndMeth=Nearest  SaturateOnIntegerOverflow=on  OutDataTypeStr=Inherit: Same as input
  b(524) : Gain  Gain=0.000129014399545789677  ParamDataTypeStr=double  RndMeth=Nearest  SaturateOnIntegerOverflow=on  OutDataTypeStr=Inherit: Same as input
  b(525) : Gain  Gain=0.000126958318748944705  ParamDataTypeStr=double  RndMeth=Nearest  SaturateOnIntegerOverflow=on  OutDataTypeStr=Inherit: Same as input
  b(526) : Gain  Gain=0.000123292979075959085  ParamDataTypeStr=double  RndMeth=Nearest  SaturateOnIntegerOverflow=on  OutDataTypeStr=Inherit: Same as input
  b(527) : Gain  Gain=0.000119600445182501628  ParamDataTypeStr=double  RndMeth=Nearest  SaturateOnIntegerOverflow=on  OutDataTypeStr=Inherit: Same as input
  b(528) : Gain  Gain=0.0013189957886183244  ParamDataTypeStr=double  RndMeth=Nearest  SaturateOnIntegerOverflow=on  OutDataTypeStr=Inherit: Same as input
  b(53) : Gain  Gain=-0.000397125758577358606  ParamDataTypeStr=double  RndMeth=Nearest  SaturateOnIntegerOverflow=on  OutDataTypeStr=Inherit: Same as input
  b(54) : Gain  Gain=-0.000391841892495430836  ParamDataTypeStr=double  RndMeth=Nearest  SaturateOnIntegerOverflow=on  OutDataTypeStr=Inherit: Same as input
  b(55) : Gain  Gain=-0.000385359957846202793  ParamDataTypeStr=double  RndMeth=Nearest  SaturateOnIntegerOverflow=on  OutDataTypeStr=Inherit: Same as input
  b(56) : Gain  Gain=-0.000376818546642253716  ParamDataTypeStr=double  RndMeth=Nearest  SaturateOnIntegerOverflow=on  OutDataTypeStr=Inherit: Same as input
  b(57) : Gain  Gain=-0.000367171401728139373  ParamDataTypeStr=double  RndMeth=Nearest  SaturateOnIntegerOverflow=on  OutDataTypeStr=Inherit: Same as input
  b(58) : Gain  Gain=-0.000355511706333689866  ParamDataTypeStr=double  RndMeth=Nearest  SaturateOnIntegerOverflow=on  OutDataTypeStr=Inherit: Same as input
  b(59) : Gain  Gain=-0.000342894954706609613  ParamDataTypeStr=double  RndMeth=Nearest  SaturateOnIntegerOverflow=on  OutDataTypeStr=Inherit: Same as input
  b(6) : Gain  Gain=0.000131022132570349182  ParamDataTypeStr=double  RndMeth=Nearest  SaturateOnIntegerOverflow=on  OutDataTypeStr=Inherit: Same as input
  b(60) : Gain  Gain=-0.000328612037461096336  ParamDataTypeStr=double  RndMeth=Nearest  SaturateOnIntegerOverflow=on  OutDataTypeStr=Inherit: Same as input
  b(61) : Gain  Gain=-0.000313697423958395668  ParamDataTypeStr=double  RndMeth=Nearest  SaturateOnIntegerOverflow=on  OutDataTypeStr=Inherit: Same as input
  b(62) : Gain  Gain=-0.000296990192063201945  ParamDataTypeStr=double  RndMeth=Nearest  SaturateOnIntegerOverflow=on  OutDataTypeStr=Inherit: Same as input
  b(63) : Gain  Gain=-0.000280071574432796044  ParamDataTypeStr=double  RndMeth=Nearest  SaturateOnIntegerOverflow=on  OutDataTypeStr=Inherit: Same as input
  b(64) : Gain  Gain=-0.000261789142866730284  ParamDataTypeStr=double  RndMeth=Nearest  SaturateOnIntegerOverflow=on  OutDataTypeStr=Inherit: Same as input
  b(65) : Gain  Gain=-0.000243411438438570623  ParamDataTypeStr=double  RndMeth=Nearest  SaturateOnIntegerOverflow=on  OutDataTypeStr=Inherit: Same as input
  b(66) : Gain  Gain=-0.00022414279328602355  ParamDataTypeStr=double  RndMeth=Nearest  SaturateOnIntegerOverflow=on  OutDataTypeStr=Inherit: Same as input
  b(67) : Gain  Gain=-0.00020509011935799723  ParamDataTypeStr=double  RndMeth=Nearest  SaturateOnIntegerOverflow=on  OutDataTypeStr=Inherit: Same as input
  b(68) : Gain  Gain=-0.000185503270808741157  ParamDataTypeStr=double  RndMeth=Nearest  SaturateOnIntegerOverflow=on  OutDataTypeStr=Inherit: Same as input
  b(69) : Gain  Gain=-0.000166478229983800735  ParamDataTypeStr=double  RndMeth=Nearest  SaturateOnIntegerOverflow=on  OutDataTypeStr=Inherit: Same as input
  b(7) : Gain  Gain=0.000131388393933855882  ParamDataTypeStr=double  RndMeth=Nearest  SaturateOnIntegerOverflow=on  OutDataTypeStr=Inherit: Same as input
  b(70) : Gain  Gain=-0.000147315132967771201  ParamDataTypeStr=double  RndMeth=Nearest  SaturateOnIntegerOverflow=on  OutDataTypeStr=Inherit: Same as input
  b(71) : Gain  Gain=-0.000129141873349178935  ParamDataTypeStr=double  RndMeth=Nearest  SaturateOnIntegerOverflow=on  OutDataTypeStr=Inherit: Same as input
  b(72) : Gain  Gain=-0.00011125252133578384  ParamDataTypeStr=double  RndMeth=Nearest  SaturateOnIntegerOverflow=on  OutDataTypeStr=Inherit: Same as input
  b(73) : Gain  Gain=-9.46829036739340896e-05  ParamDataTypeStr=double  RndMeth=Nearest  SaturateOnIntegerOverflow=on  OutDataTypeStr=Inherit: Same as input
  b(74) : Gain  Gain=-7.87286212535760581e-05  ParamDataTypeStr=double  RndMeth=Nearest  SaturateOnIntegerOverflow=on  OutDataTypeStr=Inherit: Same as input
  b(75) : Gain  Gain=-6.45312083203074521e-05  ParamDataTypeStr=double  RndMeth=Nearest  SaturateOnIntegerOverflow=on  OutDataTypeStr=Inherit: Same as input
  b(76) : Gain  Gain=-5.15015329802558704e-05  ParamDataTypeStr=double  RndMeth=Nearest  SaturateOnIntegerOverflow=on  OutDataTypeStr=Inherit: Same as input
  b(77) : Gain  Gain=-4.04269010002347978e-05  ParamDataTypeStr=double  RndMeth=Nearest  SaturateOnIntegerOverflow=on  OutDataTypeStr=Inherit: Same as input
  b(78) : Gain  Gain=-3.08383793457291371e-05  ParamDataTypeStr=double  RndMeth=Nearest  SaturateOnIntegerOverflow=on  OutDataTypeStr=Inherit: Same as input
  b(79) : Gain  Gain=-2.36957211731823793e-05  ParamDataTypeStr=double  RndMeth=Nearest  SaturateOnIntegerOverflow=on  OutDataTypeStr=Inherit: Same as input
  b(8) : Gain  Gain=0.000131740041189622225  ParamDataTypeStr=double  RndMeth=Nearest  SaturateOnIntegerOverflow=on  OutDataTypeStr=Inherit: Same as input
  b(80) : Gain  Gain=-1.82129216426999644e-05  ParamDataTypeStr=double  RndMeth=Nearest  SaturateOnIntegerOverflow=on  OutDataTypeStr=Inherit: Same as input
  b(81) : Gain  Gain=-1.55128158049954671e-05  ParamDataTypeStr=double  RndMeth=Nearest  SaturateOnIntegerOverflow=on  OutDataTypeStr=Inherit: Same as input
  b(82) : Gain  Gain=-1.47437363230819383e-05  ParamDataTypeStr=double  RndMeth=Nearest  SaturateOnIntegerOverflow=on  OutDataTypeStr=Inherit: Same as input
  b(83) : Gain  Gain=-1.69628308546508448e-05  ParamDataTypeStr=double  RndMeth=Nearest  SaturateOnIntegerOverflow=on  OutDataTypeStr=Inherit: Same as input
  b(84) : Gain  Gain=-2.12850613980476808e-05  ParamDataTypeStr=double  RndMeth=Nearest  SaturateOnIntegerOverflow=on  OutDataTypeStr=Inherit: Same as input
  b(85) : Gain  Gain=-2.87166278037361087e-05  ParamDataTypeStr=double  RndMeth=Nearest  SaturateOnIntegerOverflow=on  OutDataTypeStr=Inherit: Same as input
  b(86) : Gain  Gain=-3.83862678230118774e-05  ParamDataTypeStr=double  RndMeth=Nearest  SaturateOnIntegerOverflow=on  OutDataTypeStr=Inherit: Same as input
  b(87) : Gain  Gain=-5.127065973762235e-05  ParamDataTypeStr=double  RndMeth=Nearest  SaturateOnIntegerOverflow=on  OutDataTypeStr=Inherit: Same as input
  b(88) : Gain  Gain=-6.63999170443811595e-05  ParamDataTypeStr=double  RndMeth=Nearest  SaturateOnIntegerOverflow=on  OutDataTypeStr=Inherit: Same as input
  b(89) : Gain  Gain=-8.46336706624266095e-05  ParamDataTypeStr=double  RndMeth=Nearest  SaturateOnIntegerOverflow=on  OutDataTypeStr=Inherit: Same as input
  b(9) : Gain  Gain=0.000130387945813979691  ParamDataTypeStr=double  RndMeth=Nearest  SaturateOnIntegerOverflow=on  OutDataTypeStr=Inherit: Same as input
  b(90) : Gain  Gain=-0.000104999200466021321  ParamDataTypeStr=double  RndMeth=Nearest  SaturateOnIntegerOverflow=on  OutDataTypeStr=Inherit: Same as input
  b(91) : Gain  Gain=-0.00012844573614923015  ParamDataTypeStr=double  RndMeth=Nearest  SaturateOnIntegerOverflow=on  OutDataTypeStr=Inherit: Same as input
  b(92) : Gain  Gain=-0.000153800533059332729  ParamDataTypeStr=double  RndMeth=Nearest  SaturateOnIntegerOverflow=on  OutDataTypeStr=Inherit: Same as input
  b(93) : Gain  Gain=-0.00018187967171705505  ParamDataTypeStr=double  RndMeth=Nearest  SaturateOnIntegerOverflow=on  OutDataTypeStr=Inherit: Same as input
  b(94) : Gain  Gain=-0.000211695078287365548  ParamDataTypeStr=double  RndMeth=Nearest  SaturateOnIntegerOverflow=on  OutDataTypeStr=Inherit: Same as input
  b(95) : Gain  Gain=-0.000243803841427045562  ParamDataTypeStr=double  RndMeth=Nearest  SaturateOnIntegerOverflow=on  OutDataTypeStr=Inherit: Same as input
  b(96) : Gain  Gain=-0.00027723555258353798  ParamDataTypeStr=double  RndMeth=Nearest  SaturateOnIntegerOverflow=on  OutDataTypeStr=Inherit: Same as input
  b(97) : Gain  Gain=-0.000312529436229563081  ParamDataTypeStr=double  RndMeth=Nearest  SaturateOnIntegerOverflow=on  OutDataTypeStr=Inherit: Same as input
  b(98) : Gain  Gain=-0.000348624240333695939  ParamDataTypeStr=double  RndMeth=Nearest  SaturateOnIntegerOverflow=on  OutDataTypeStr=Inherit: Same as input
  b(99) : Gain  Gain=-0.000386007594417995138  ParamDataTypeStr=double  RndMeth=Nearest  SaturateOnIntegerOverflow=on  OutDataTypeStr=Inherit: Same as input
  Output : Outport
  wires:
  Input/1 -> b(1)/1, BodyDelay2/1
  b(1)/1 -> BodyLSum2/2
  BodyDelay2/1 -> b(2)/1, BodyDelay3/1
  b(2)/1 -> BodyLSum2/1
  BodyLSum2/1 -> BodyLSum3/2
  BodyDelay3/1 -> b(3)/1, BodyDelay4/1
  b(3)/1 -> BodyLSum3/1
  BodyLSum3/1 -> BodyLSum4/2
  BodyDelay4/1 -> b(4)/1, BodyDelay5/1
  b(4)/1 -> BodyLSum4/1
  BodyLSum4/1 -> BodyLSum5/2
  BodyDelay5/1 -> b(5)/1, BodyDelay6/1
  b(5)/1 -> BodyLSum5/1
  BodyLSum5/1 -> BodyLSum6/2
  BodyDelay6/1 -> b(6)/1, BodyDelay7/1
  b(6)/1 -> BodyLSum6/1
  BodyLSum6/1 -> BodyLSum7/2
  BodyDelay7/1 -> b(7)/1, BodyDelay8/1
  b(7)/1 -> BodyLSum7/1
  BodyLSum7/1 -> BodyLSum8/2
  BodyDelay8/1 -> b(8)/1, BodyDelay9/1
  b(8)/1 -> BodyLSum8/1
  BodyLSum8/1 -> BodyLSum9/2
  BodyDelay9/1 -> b(9)/1, BodyDelay10/1
  b(9)/1 -> BodyLSum9/1
  BodyLSum9/1 -> BodyLSum10/2
  BodyDelay10/1 -> b(10)/1, BodyDelay11/1
  b(10)/1 -> BodyLSum10/1
  BodyLSum10/1 -> BodyLSum11/2
  BodyDelay11/1 -> b(11)/1, BodyDelay12/1
  b(11)/1 -> BodyLSum11/1
  BodyLSum11/1 -> BodyLSum12/2
  BodyDelay12/1 -> b(12)/1, BodyDelay13/1
  b(12)/1 -> BodyLSum12/1
  BodyLSum12/1 -> BodyLSum13/2
  BodyDelay13/1 -> b(13)/1, BodyDelay14/1
  b(13)/1 -> BodyLSum13/1
  BodyLSum13/1 -> BodyLSum14/2
  BodyDelay14/1 -> b(14)/1, BodyDelay15/1
  b(14)/1 -> BodyLSum14/1
  BodyLSum14/1 -> BodyLSum15/2
  BodyDelay15/1 -> b(15)/1, BodyDelay16/1
  b(15)/1 -> BodyLSum15/1
  BodyLSum15/1 -> BodyLSum16/2
  BodyDelay16/1 -> b(16)/1, BodyDelay17/1
  b(16)/1 -> BodyLSum16/1
  BodyLSum16/1 -> BodyLSum17/2
  BodyDelay17/1 -> b(17)/1, BodyDelay18/1
  b(17)/1 -> BodyLSum17/1
  BodyLSum17/1 -> BodyLSum18/2
  BodyDelay18/1 -> b(18)/1, BodyDelay19/1
  b(18)/1 -> BodyLSum18/1
  BodyLSum18/1 -> BodyLSum19/2
  BodyDelay19/1 -> b(19)/1, BodyDelay20/1
  b(19)/1 -> BodyLSum19/1
  BodyLSum19/1 -> BodyLSum20/2
  BodyDelay20/1 -> b(20)/1, BodyDelay21/1
  b(20)/1 -> BodyLSum20/1
  BodyLSum20/1 -> BodyLSum21/2
  BodyDelay21/1 -> b(21)/1, BodyDelay22/1
  b(21)/1 -> BodyLSum21/1
  BodyLSum21/1 -> BodyLSum22/2
  BodyDelay22/1 -> b(22)/1, BodyDelay23/1
  b(22)/1 -> BodyLSum22/1
  BodyLSum22/1 -> BodyLSum23/2
  BodyDelay23/1 -> b(23)/1, BodyDelay24/1
  b(23)/1 -> BodyLSum23/1
  BodyLSum23/1 -> BodyLSum24/2
  BodyDelay24/1 -> b(24)/1, BodyDelay25/1
  b(24)/1 -> BodyLSum24/1
  BodyLSum24/1 -> BodyLSum25/2
  BodyDelay25/1 -> b(25)/1, BodyDelay26/1
  b(25)/1 -> BodyLSum25/1
  BodyLSum25/1 -> BodyLSum26/2
  BodyDelay26/1 -> b(26)/1, BodyDelay27/1
  b(26)/1 -> BodyLSum26/1
  BodyLSum26/1 -> BodyLSum27/2
  BodyDelay27/1 -> b(27)/1, BodyDelay28/1
  b(27)/1 -> BodyLSum27/1
  BodyLSum27/1 -> BodyLSum28/2
  BodyDelay28/1 -> b(28)/1, BodyDelay29/1
  b(28)/1 -> BodyLSum28/1
  BodyLSum28/1 -> BodyLSum29/2
  BodyDelay29/1 -> b(29)/1, BodyDelay30/1
  b(29)/1 -> BodyLSum29/1
  BodyLSum29/1 -> BodyLSum30/2
  BodyDelay30/1 -> b(30)/1, BodyDelay31/1
  b(30)/1 -> BodyLSum30/1
  BodyLSum30/1 -> BodyLSum31/2
  BodyDelay31/1 -> b(31)/1, BodyDelay32/1
  b(31)/1 -> BodyLSum31/1
  BodyLSum31/1 -> BodyLSum32/2
  BodyDelay32/1 -> b(32)/1, BodyDelay33/1
  b(32)/1 -> BodyLSum32/1
  BodyLSum32/1 -> BodyLSum33/2
  BodyDelay33/1 -> b(33)/1, BodyDelay34/1
  b(33)/1 -> BodyLSum33/1
  BodyLSum33/1 -> BodyLSum34/2
  BodyDelay34/1 -> b(34)/1, BodyDelay35/1
  b(34)/1 -> BodyLSum34/1
  BodyLSum34/1 -> BodyLSum35/2
  BodyDelay35/1 -> b(35)/1, BodyDelay36/1
  b(35)/1 -> BodyLSum35/1
  BodyLSum35/1 -> BodyLSum36/2
  BodyDelay36/1 -> b(36)/1, BodyDelay37/1
  b(36)/1 -> BodyLSum36/1
  BodyLSum36/1 -> BodyLSum37/2
  BodyDelay37/1 -> b(37)/1, BodyDelay38/1
  b(37)/1 -> BodyLSum37/1
  BodyLSum37/1 -> BodyLSum38/2
  BodyDelay38/1 -> b(38)/1, BodyDelay39/1
  b(38)/1 -> BodyLSum38/1
  BodyLSum38/1 -> BodyLSum39/2
  BodyDelay39/1 -> b(39)/1, BodyDelay40/1
  b(39)/1 -> BodyLSum39/1
  BodyLSum39/1 -> BodyLSum40/2
  BodyDelay40/1 -> b(40)/1, BodyDelay41/1
  b(40)/1 -> BodyLSum40/1
  BodyLSum40/1 -> BodyLSum41/2
  BodyDelay41/1 -> b(41)/1, BodyDelay42/1
  b(41)/1 -> BodyLSum41/1
  BodyLSum41/1 -> BodyLSum42/2
  BodyDelay42/1 -> b(42)/1, BodyDelay43/1
  b(42)/1 -> BodyLSum42/1
  BodyLSum42/1 -> BodyLSum43/2
  BodyDelay43/1 -> b(43)/1, BodyDelay44/1
  b(43)/1 -> BodyLSum43/1
  BodyLSum43/1 -> BodyLSum44/2
  BodyDelay44/1 -> b(44)/1, BodyDelay45/1
  b(44)/1 -> BodyLSum44/1
  BodyLSum44/1 -> BodyLSum45/2
  BodyDelay45/1 -> b(45)/1, BodyDelay46/1
  b(45)/1 -> BodyLSum45/1
  BodyLSum45/1 -> BodyLSum46/2
  BodyDelay46/1 -> b(46)/1, BodyDelay47/1
  b(46)/1 -> BodyLSum46/1
  BodyLSum46/1 -> BodyLSum47/2
  BodyDelay47/1 -> b(47)/1, BodyDelay48/1
  b(47)/1 -> BodyLSum47/1
  BodyLSum47/1 -> BodyLSum48/2
  BodyDelay48/1 -> b(48)/1, BodyDelay49/1
  b(48)/1 -> BodyLSum48/1
  BodyLSum48/1 -> BodyLSum49/2
  BodyDelay49/1 -> b(49)/1, BodyDelay50/1
  b(49)/1 -> BodyLSum49/1
  BodyLSum49/1 -> BodyLSum50/2
  BodyDelay50/1 -> b(50)/1, BodyDelay51/1
  b(50)/1 -> BodyLSum50/1
  BodyLSum50/1 -> BodyLSum51/2
  BodyDelay51/1 -> b(51)/1, BodyDelay52/1
  b(51)/1 -> BodyLSum51/1
  BodyLSum51/1 -> BodyLSum52/2
  BodyDelay52/1 -> b(52)/1, BodyDelay53/1
  b(52)/1 -> BodyLSum52/1
  BodyLSum52/1 -> BodyLSum53/2
  BodyDelay53/1 -> b(53)/1, BodyDelay54/1
  b(53)/1 -> BodyLSum53/1
  BodyLSum53/1 -> BodyLSum54/2
  BodyDelay54/1 -> b(54)/1, BodyDelay55/1
  b(54)/1 -> BodyLSum54/1
  BodyLSum54/1 -> BodyLSum55/2
  BodyDelay55/1 -> b(55)/1, BodyDelay56/1
  b(55)/1 -> BodyLSum55/1
  BodyLSum55/1 -> BodyLSum56/2
  BodyDelay56/1 -> b(56)/1, BodyDelay57/1
  b(56)/1 -> BodyLSum56/1
  BodyLSum56/1 -> BodyLSum57/2
  BodyDelay57/1 -> b(57)/1, BodyDelay58/1
  b(57)/1 -> BodyLSum57/1
  BodyLSum57/1 -> BodyLSum58/2
  BodyDelay58/1 -> b(58)/1, BodyDelay59/1
  b(58)/1 -> BodyLSum58/1
  BodyLSum58/1 -> BodyLSum59/2
  BodyDelay59/1 -> b(59)/1, BodyDelay60/1
  b(59)/1 -> BodyLSum59/1
  BodyLSum59/1 -> BodyLSum60/2
  BodyDelay60/1 -> b(60)/1, BodyDelay61/1
  b(60)/1 -> BodyLSum60/1
  BodyLSum60/1 -> BodyLSum61/2
  BodyDelay61/1 -> b(61)/1, BodyDelay62/1
  b(61)/1 -> BodyLSum61/1
  BodyLSum61/1 -> BodyLSum62/2
  BodyDelay62/1 -> b(62)/1, BodyDelay63/1
  b(62)/1 -> BodyLSum62/1
  BodyLSum62/1 -> BodyLSum63/2
  BodyDelay63/1 -> b(63)/1, BodyDelay64/1
  b(63)/1 -> BodyLSum63/1
  BodyLSum63/1 -> BodyLSum64/2
  BodyDelay64/1 -> b(64)/1, BodyDelay65/1
  b(64)/1 -> BodyLSum64/1
  BodyLSum64/1 -> BodyLSum65/2
  BodyDelay65/1 -> b(65)/1, BodyDelay66/1
  b(65)/1 -> BodyLSum65/1
  BodyLSum65/1 -> BodyLSum66/2
  BodyDelay66/1 -> b(66)/1, BodyDelay67/1
  b(66)/1 -> BodyLSum66/1
  BodyLSum66/1 -> BodyLSum67/2
  BodyDelay67/1 -> b(67)/1, BodyDelay68/1
  b(67)/1 -> BodyLSum67/1
  BodyLSum67/1 -> BodyLSum68/2
  BodyDelay68/1 -> b(68)/1, BodyDelay69/1
  b(68)/1 -> BodyLSum68/1
  BodyLSum68/1 -> BodyLSum69/2
  BodyDelay69/1 -> b(69)/1, BodyDelay70/1
  b(69)/1 -> BodyLSum69/1
  BodyLSum69/1 -> BodyLSum70/2
  BodyDelay70/1 -> b(70)/1, BodyDelay71/1
  b(70)/1 -> BodyLSum70/1
  BodyLSum70/1 -> BodyLSum71/2
  BodyDelay71/1 -> b(71)/1, BodyDelay72/1
  b(71)/1 -> BodyLSum71/1
  BodyLSum71/1 -> BodyLSum72/2
  BodyDelay72/1 -> b(72)/1, BodyDelay73/1
  b(72)/1 -> BodyLSum72/1
  BodyLSum72/1 -> BodyLSum73/2
  BodyDelay73/1 -> b(73)/1, BodyDelay74/1
  b(73)/1 -> BodyLSum73/1
  BodyLSum73/1 -> BodyLSum74/2
  BodyDelay74/1 -> b(74)/1, BodyDelay75/1
  b(74)/1 -> BodyLSum74/1
  BodyLSum74/1 -> BodyLSum75/2
  BodyDelay75/1 -> b(75)/1, BodyDelay76/1
  b(75)/1 -> BodyLSum75/1
  BodyLSum75/1 -> BodyLSum76/2
  BodyDelay76/1 -> b(76)/1, BodyDelay77/1
  b(76)/1 -> BodyLSum76/1
  BodyLSum76/1 -> BodyLSum77/2
  BodyDelay77/1 -> b(77)/1, BodyDelay78/1
  b(77)/1 -> BodyLSum77/1
  BodyLSum77/1 -> BodyLSum78/2
  BodyDelay78/1 -> b(78)/1, BodyDelay79/1
  b(78)/1 -> BodyLSum78/1
  BodyLSum78/1 -> BodyLSum79/2
  BodyDelay79/1 -> b(79)/1, BodyDelay80/1
  b(79)/1 -> BodyLSum79/1
  BodyLSum79/1 -> BodyLSum80/2
  BodyDelay80/1 -> b(80)/1, BodyDelay81/1
  b(80)/1 -> BodyLSum80/1
  BodyLSum80/1 -> BodyLSum81/2
  BodyDelay81/1 -> b(81)/1, BodyDelay82/1
  b(81)/1 -> BodyLSum81/1
  BodyLSum81/1 -> BodyLSum82/2
  BodyDelay82/1 -> b(82)/1, BodyDelay83/1
  b(82)/1 -> BodyLSum82/1
  BodyLSum82/1 -> BodyLSum83/2
  BodyDelay83/1 -> b(83)/1, BodyDelay84/1
  b(83)/1 -> BodyLSum83/1
  BodyLSum83/1 -> BodyLSum84/2
  BodyDelay84/1 -> b(84)/1, BodyDelay85/1
  b(84)/1 -> BodyLSum84/1
  BodyLSum84/1 -> BodyLSum85/2
  BodyDelay85/1 -> b(85)/1, BodyDelay86/1
  b(85)/1 -> BodyLSum85/1
  BodyLSum85/1 -> BodyLSum86/2
  BodyDelay86/1 -> b(86)/1, BodyDelay87/1
  b(86)/1 -> BodyLSum86/1
  BodyLSum86/1 -> BodyLSum87/2
  BodyDelay87/1 -> b(87)/1, BodyDelay88/1
  b(87)/1 -> BodyLSum87/1
  BodyLSum87/1 -> BodyLSum88/2
  BodyDelay88/1 -> b(88)/1, BodyDelay89/1
  b(88)/1 -> BodyLSum88/1
  BodyLSum88/1 -> BodyLSum89/2
  BodyDelay89/1 -> b(89)/1, BodyDelay90/1
  b(89)/1 -> BodyLSum89/1
  BodyLSum89/1 -> BodyLSum90/2
  BodyDelay90/1 -> b(90)/1, BodyDelay91/1
  b(90)/1 -> BodyLSum90/1
  BodyLSum90/1 -> BodyLSum91/2
  BodyDelay91/1 -> b(91)/1, BodyDelay92/1
  b(91)/1 -> BodyLSum91/1
  BodyLSum91/1 -> BodyLSum92/2
  BodyDelay92/1 -> b(92)/1, BodyDelay93/1
  b(92)/1 -> BodyLSum92/1
  BodyLSum92/1 -> BodyLSum93/2
  BodyDelay93/1 -> b(93)/1, BodyDelay94/1
  b(93)/1 -> BodyLSum93/1
  BodyLSum93/1 -> BodyLSum94/2
  BodyDelay94/1 -> b(94)/1, BodyDelay95/1
  b(94)/1 -> BodyLSum94/1
  BodyLSum94/1 -> BodyLSum95/2
  BodyDelay95/1 -> b(95)/1, BodyDelay96/1
  b(95)/1 -> BodyLSum95/1
  BodyLSum95/1 -> BodyLSum96/2
  BodyDelay96/1 -> b(96)/1, BodyDelay97/1
  b(96)/1 -> BodyLSum96/1
  BodyLSum96/1 -> BodyLSum97/2
  BodyDelay97/1 -> b(97)/1, BodyDelay98/1
  b(97)/1 -> BodyLSum97/1
  BodyLSum97/1 -> BodyLSum98/2
  BodyDelay98/1 -> b(98)/1, BodyDelay99/1
  b(98)/1 -> BodyLSum98/1
  BodyLSum98/1 -> BodyLSum99/2
  BodyDelay99/1 -> b(99)/1, BodyDelay100/1
  b(99)/1 -> BodyLSum99/1
  BodyLSum99/1 -> BodyLSum100/2
  BodyDelay100/1 -> b(100)/1, BodyDelay101/1
  b(100)/1 -> BodyLSum100/1
  BodyLSum100/1 -> BodyLSum101/2
  BodyDelay101/1 -> b(101)/1, BodyDelay102/1
  b(101)/1 -> BodyLSum101/1
  BodyLSum101/1 -> BodyLSum102/2
  BodyDelay102/1 -> b(102)/1, BodyDelay103/1
  b(102)/1 -> BodyLSum102/1
  BodyLSum102/1 -> BodyLSum103/2
  BodyDelay103/1 -> b(103)/1, BodyDelay104/1
  b(103)/1 -> BodyLSum103/1
  BodyLSum103/1 -> BodyLSum104/2
  BodyDelay104/1 -> b(104)/1, BodyDelay105/1
  b(104)/1 -> BodyLSum104/1
  BodyLSum104/1 -> BodyLSum105/2
  BodyDelay105/1 -> b(105)/1, BodyDelay106/1
  b(105)/1 -> BodyLSum105/1
  BodyLSum105/1 -> BodyLSum106/2
  BodyDelay106/1 -> b(106)/1, BodyDelay107/1
  b(106)/1 -> BodyLSum106/1
  BodyLSum106/1 -> BodyLSum107/2
  BodyDelay107/1 -> b(107)/1, BodyDelay108/1
  b(107)/1 -> BodyLSum107/1
  BodyLSum107/1 -> BodyLSum108/2
  BodyDelay108/1 -> b(108)/1, BodyDelay109/1
  b(108)/1 -> BodyLSum108/1
  BodyLSum108/1 -> BodyLSum109/2
  BodyDelay109/1 -> b(109)/1, BodyDelay110/1
  b(109)/1 -> BodyLSum109/1
  BodyLSum109/1 -> BodyLSum110/2
  BodyDelay110/1 -> b(110)/1, BodyDelay111/1
  b(110)/1 -> BodyLSum110/1
  BodyLSum110/1 -> BodyLSum111/2
  BodyDelay111/1 -> b(111)/1, BodyDelay112/1
  b(111)/1 -> BodyLSum111/1
  BodyLSum111/1 -> BodyLSum112/2
  BodyDelay112/1 -> b(112)/1, BodyDelay113/1
  b(112)/1 -> BodyLSum112/1
  BodyLSum112/1 -> BodyLSum113/2
  BodyDelay113/1 -> b(113)/1, BodyDelay114/1
  b(113)/1 -> BodyLSum113/1
  BodyLSum113/1 -> BodyLSum114/2
  BodyDelay114/1 -> b(114)/1, BodyDelay115/1
  b(114)/1 -> BodyLSum114/1
  BodyLSum114/1 -> BodyLSum115/2
  BodyDelay115/1 -> b(115)/1, BodyDelay116/1
  b(115)/1 -> BodyLSum115/1
  BodyLSum115/1 -> BodyLSum116/2
  BodyDelay116/1 -> b(116)/1, BodyDelay117/1
  b(116)/1 -> BodyLSum116/1
  BodyLSum116/1 -> BodyLSum117/2
  BodyDelay117/1 -> b(117)/1, BodyDelay118/1
  b(117)/1 -> BodyLSum117/1
  BodyLSum117/1 -> BodyLSum118/2
  BodyDelay118/1 -> b(118)/1, BodyDelay119/1
  b(118)/1 -> BodyLSum118/1
  BodyLSum118/1 -> BodyLSum119/2
  BodyDelay119/1 -> b(119)/1, BodyDelay120/1
  b(119)/1 -> BodyLSum119/1
  BodyLSum119/1 -> BodyLSum120/2
  BodyDelay120/1 -> b(120)/1, BodyDelay121/1
  b(120)/1 -> BodyLSum120/1
  BodyLSum120/1 -> BodyLSum121/2
  BodyDelay121/1 -> b(121)/1, BodyDelay122/1
  b(121)/1 -> BodyLSum121/1
  BodyLSum121/1 -> BodyLSum122/2
  BodyDelay122/1 -> b(122)/1, BodyDelay123/1
  b(122)/1 -> BodyLSum122/1
  BodyLSum122/1 -> BodyLSum123/2
  BodyDelay123/1 -> b(123)/1, BodyDelay124/1
  b(123)/1 -> BodyLSum123/1
  BodyLSum123/1 -> BodyLSum124/2
  BodyDelay124/1 -> b(124)/1, BodyDelay125/1
  b(124)/1 -> BodyLSum124/1
  BodyLSum124/1 -> BodyLSum125/2
  BodyDelay125/1 -> b(125)/1, BodyDelay126/1
  b(125)/1 -> BodyLSum125/1
  BodyLSum125/1 -> BodyLSum126/2
  BodyDelay126/1 -> b(126)/1, BodyDelay127/1
  b(126)/1 -> BodyLSum126/1
  BodyLSum126/1 -> BodyLSum127/2
  BodyDelay127/1 -> b(127)/1, BodyDelay128/1
  b(127)/1 -> BodyLSum127/1
  BodyLSum127/1 -> BodyLSum128/2
  BodyDelay128/1 -> b(128)/1, BodyDelay129/1
  b(128)/1 -> BodyLSum128/1
  BodyLSum128/1 -> BodyLSum129/2
  BodyDelay129/1 -> b(129)/1, BodyDelay130/1
  b(129)/1 -> BodyLSum129/1
  BodyLSum129/1 -> BodyLSum130/2
  BodyDelay130/1 -> b(130)/1, BodyDelay131/1
  b(130)/1 -> BodyLSum130/1
  BodyLSum130/1 -> BodyLSum131/2
  BodyDelay131/1 -> b(131)/1, BodyDelay132/1
  b(131)/1 -> BodyLSum131/1
  BodyLSum131/1 -> BodyLSum132/2
  BodyDelay132/1 -> b(132)/1, BodyDelay133/1
  b(132)/1 -> BodyLSum132/1
  BodyLSum132/1 -> BodyLSum133/2
  BodyDelay133/1 -> b(133)/1, BodyDelay134/1
  b(133)/1 -> BodyLSum133/1
  BodyLSum133/1 -> BodyLSum134/2
  BodyDelay134/1 -> b(134)/1, BodyDelay135/1
  b(134)/1 -> BodyLSum134/1
  BodyLSum134/1 -> BodyLSum135/2
  BodyDelay135/1 -> b(135)/1, BodyDelay136/1
  b(135)/1 -> BodyLSum135/1
  BodyLSum135/1 -> BodyLSum136/2
  BodyDelay136/1 -> b(136)/1, BodyDelay137/1
  b(136)/1 -> BodyLSum136/1
  BodyLSum136/1 -> BodyLSum137/2
  BodyDelay137/1 -> b(137)/1, BodyDelay138/1
  b(137)/1 -> BodyLSum137/1
  BodyLSum137/1 -> BodyLSum138/2
  BodyDelay138/1 -> b(138)/1, BodyDelay139/1
  b(138)/1 -> BodyLSum138/1
  BodyLSum138/1 -> BodyLSum139/2
  BodyDelay139/1 -> b(139)/1, BodyDelay140/1
  b(139)/1 -> BodyLSum139/1
  BodyLSum139/1 -> BodyLSum140/2
  BodyDelay140/1 -> b(140)/1, BodyDelay141/1
  b(140)/1 -> BodyLSum140/1
  BodyLSum140/1 -> BodyLSum141/2
  BodyDelay141/1 -> b(141)/1, BodyDelay142/1
  b(141)/1 -> BodyLSum141/1
  BodyLSum141/1 -> BodyLSum142/2
  BodyDelay142/1 -> b(142)/1, BodyDelay143/1
  b(142)/1 -> BodyLSum142/1
  BodyLSum142/1 -> BodyLSum143/2
  BodyDelay143/1 -> b(143)/1, BodyDelay144/1
  b(143)/1 -> BodyLSum143/1
  BodyLSum143/1 -> BodyLSum144/2
  BodyDelay144/1 -> b(144)/1, BodyDelay145/1
  b(144)/1 -> BodyLSum144/1
  BodyLSum144/1 -> BodyLSum145/2
  BodyDelay145/1 -> b(145)/1, BodyDelay146/1
  b(145)/1 -> BodyLSum145/1
  BodyLSum145/1 -> BodyLSum146/2
  BodyDelay146/1 -> b(146)/1, BodyDelay147/1
  b(146)/1 -> BodyLSum146/1
  BodyLSum146/1 -> BodyLSum147/2
  BodyDelay147/1 -> b(147)/1, BodyDelay148/1
  b(147)/1 -> BodyLSum147/1
  BodyLSum147/1 -> BodyLSum148/2
  BodyDelay148/1 -> b(148)/1, BodyDelay149/1
  b(148)/1 -> BodyLSum148/1
  BodyLSum148/1 -> BodyLSum149/2
  BodyDelay149/1 -> b(149)/1, BodyDelay150/1
  b(149)/1 -> BodyLSum149/1
  BodyLSum149/1 -> BodyLSum150/2
  BodyDelay150/1 -> b(150)/1, BodyDelay151/1
  b(150)/1 -> BodyLSum150/1
  BodyLSum150/1 -> BodyLSum151/2
  BodyDelay151/1 -> b(151)/1, BodyDelay152/1
  b(151)/1 -> BodyLSum151/1
  BodyLSum151/1 -> BodyLSum152/2
  BodyDelay152/1 -> b(152)/1, BodyDelay153/1
  b(152)/1 -> BodyLSum152/1
  BodyLSum152/1 -> BodyLSum153/2
  BodyDelay153/1 -> b(153)/1, BodyDelay154/1
  b(153)/1 -> BodyLSum153/1
  BodyLSum153/1 -> BodyLSum154/2
  BodyDelay154/1 -> b(154)/1, BodyDelay155/1
  b(154)/1 -> BodyLSum154/1
  BodyLSum154/1 -> BodyLSum155/2
  BodyDelay155/1 -> b(155)/1, BodyDelay156/1
  b(155)/1 -> BodyLSum155/1
  BodyLSum155/1 -> BodyLSum156/2
  BodyDelay156/1 -> b(156)/1, BodyDelay157/1
  b(156)/1 -> BodyLSum156/1
  BodyLSum156/1 -> BodyLSum157/2
  BodyDelay157/1 -> b(157)/1, BodyDelay158/1
  b(157)/1 -> BodyLSum157/1
  BodyLSum157/1 -> BodyLSum158/2
  BodyDelay158/1 -> b(158)/1, BodyDelay159/1
  b(158)/1 -> BodyLSum158/1
  BodyLSum158/1 -> BodyLSum159/2
  BodyDelay159/1 -> b(159)/1, BodyDelay160/1
  b(159)/1 -> BodyLSum159/1
  BodyLSum159/1 -> BodyLSum160/2
  BodyDelay160/1 -> b(160)/1, BodyDelay161/1
  b(160)/1 -> BodyLSum160/1
  BodyLSum160/1 -> BodyLSum161/2
  BodyDelay161/1 -> b(161)/1, BodyDelay162/1
  b(161)/1 -> BodyLSum161/1
  BodyLSum161/1 -> BodyLSum162/2
  BodyDelay162/1 -> b(162)/1, BodyDelay163/1
  b(162)/1 -> BodyLSum162/1
  BodyLSum162/1 -> BodyLSum163/2
  BodyDelay163/1 -> b(163)/1, BodyDelay164/1
  b(163)/1 -> BodyLSum163/1
  BodyLSum163/1 -> BodyLSum164/2
  BodyDelay164/1 -> b(164)/1, BodyDelay165/1
  b(164)/1 -> BodyLSum164/1
  BodyLSum164/1 -> BodyLSum165/2
  BodyDelay165/1 -> b(165)/1, BodyDelay166/1
  b(165)/1 -> BodyLSum165/1
  BodyLSum165/1 -> BodyLSum166/2
  BodyDelay166/1 -> b(166)/1, BodyDelay167/1
  b(166)/1 -> BodyLSum166/1
  BodyLSum166/1 -> BodyLSum167/2
  BodyDelay167/1 -> b(167)/1, BodyDelay168/1
  b(167)/1 -> BodyLSum167/1
  BodyLSum167/1 -> BodyLSum168/2
  BodyDelay168/1 -> b(168)/1, BodyDelay169/1
  b(168)/1 -> BodyLSum168/1
  BodyLSum168/1 -> BodyLSum169/2
  BodyDelay169/1 -> b(169)/1, BodyDelay170/1
  b(169)/1 -> BodyLSum169/1
  BodyLSum169/1 -> BodyLSum170/2
  BodyDelay170/1 -> b(170)/1, BodyDelay171/1
  b(170)/1 -> BodyLSum170/1
  BodyLSum170/1 -> BodyLSum171/2
  BodyDelay171/1 -> b(171)/1, BodyDelay172/1
  b(171)/1 -> BodyLSum171/1
  BodyLSum171/1 -> BodyLSum172/2
  BodyDelay172/1 -> b(172)/1, BodyDelay173/1
  b(172)/1 -> BodyLSum172/1
  BodyLSum172/1 -> BodyLSum173/2
  BodyDelay173/1 -> b(173)/1, BodyDelay174/1
  b(173)/1 -> BodyLSum173/1
  BodyLSum173/1 -> BodyLSum174/2
  BodyDelay174/1 -> b(174)/1, BodyDelay175/1
  b(174)/1 -> BodyLSum174/1
  BodyLSum174/1 -> BodyLSum175/2
  BodyDelay175/1 -> b(175)/1, BodyDelay176/1
  b(175)/1 -> BodyLSum175/1
  BodyLSum175/1 -> BodyLSum176/2
  BodyDelay176/1 -> b(176)/1, BodyDelay177/1
  b(176)/1 -> BodyLSum176/1
  BodyLSum176/1 -> BodyLSum177/2
  BodyDelay177/1 -> b(177)/1, BodyDelay178/1
  b(177)/1 -> BodyLSum177/1
  BodyLSum177/1 -> BodyLSum178/2
  BodyDelay178/1 -> b(178)/1, BodyDelay179/1
  b(178)/1 -> BodyLSum178/1
  BodyLSum178/1 -> BodyLSum179/2
  BodyDelay179/1 -> b(179)/1, BodyDelay180/1
  b(179)/1 -> BodyLSum179/1
  BodyLSum179/1 -> BodyLSum180/2
  BodyDelay180/1 -> b(180)/1, BodyDelay181/1
  b(180)/1 -> BodyLSum180/1
  BodyLSum180/1 -> BodyLSum181/2
  BodyDelay181/1 -> b(181)/1, BodyDelay182/1
  b(181)/1 -> BodyLSum181/1
  BodyLSum181/1 -> BodyLSum182/2
  BodyDelay182/1 -> b(182)/1, BodyDelay183/1
  b(182)/1 -> BodyLSum182/1
  BodyLSum182/1 -> BodyLSum183/2
  BodyDelay183/1 -> b(183)/1, BodyDelay184/1
  b(183)/1 -> BodyLSum183/1
  BodyLSum183/1 -> BodyLSum184/2
  BodyDelay184/1 -> b(184)/1, BodyDelay185/1
  b(184)/1 -> BodyLSum184/1
  BodyLSum184/1 -> BodyLSum185/2
  BodyDelay185/1 -> b(185)/1, BodyDelay186/1
  b(185)/1 -> BodyLSum185/1
  BodyLSum185/1 -> BodyLSum186/2
  BodyDelay186/1 -> b(186)/1, BodyDelay187/1
  b(186)/1 -> BodyLSum186/1
  BodyLSum186/1 -> BodyLSum187/2
  BodyDelay187/1 -> b(187)/1, BodyDelay188/1
  b(187)/1 -> BodyLSum187/1
  BodyLSum187/1 -> BodyLSum188/2
  BodyDelay188/1 -> b(188)/1, BodyDelay189/1
  b(188)/1 -> BodyLSum188/1
  BodyLSum188/1 -> BodyLSum189/2
  BodyDelay189/1 -> b(189)/1, BodyDelay190/1
  b(189)/1 -> BodyLSum189/1
  BodyLSum189/1 -> BodyLSum190/2
  BodyDelay190/1 -> b(190)/1, BodyDelay191/1
  b(190)/1 -> BodyLSum190/1
  BodyLSum190/1 -> BodyLSum191/2
  BodyDelay191/1 -> b(191)/1, BodyDelay192/1
  b(191)/1 -> BodyLSum191/1
  BodyLSum191/1 -> BodyLSum192/2
  BodyDelay192/1 -> b(192)/1, BodyDelay193/1
  b(192)/1 -> BodyLSum192/1
  BodyLSum192/1 -> BodyLSum193/2
  BodyDelay193/1 -> b(193)/1, BodyDelay194/1
  b(193)/1 -> BodyLSum193/1
  BodyLSum193/1 -> BodyLSum194/2
  BodyDelay194/1 -> b(194)/1, BodyDelay195/1
  b(194)/1 -> BodyLSum194/1
  BodyLSum194/1 -> BodyLSum195/2
  BodyDelay195/1 -> b(195)/1, BodyDelay196/1
  b(195)/1 -> BodyLSum195/1
  BodyLSum195/1 -> BodyLSum196/2
  BodyDelay196/1 -> b(196)/1, BodyDelay197/1
  b(196)/1 -> BodyLSum196/1
  BodyLSum196/1 -> BodyLSum197/2
  BodyDelay197/1 -> b(197)/1, BodyDelay198/1
  b(197)/1 -> BodyLSum197/1
  BodyLSum197/1 -> BodyLSum198/2
  BodyDelay198/1 -> b(198)/1, BodyDelay199/1
  b(198)/1 -> BodyLSum198/1
  BodyLSum198/1 -> BodyLSum199/2
  BodyDelay199/1 -> b(199)/1, BodyDelay200/1
  b(199)/1 -> BodyLSum199/1
  BodyLSum199/1 -> BodyLSum200/2
  BodyDelay200/1 -> b(200)/1, BodyDelay201/1
  b(200)/1 -> BodyLSum200/1
  BodyLSum200/1 -> BodyLSum201/2
  BodyDelay201/1 -> b(201)/1, BodyDelay202/1
  b(201)/1 -> BodyLSum201/1
  BodyLSum201/1 -> BodyLSum202/2
  BodyDelay202/1 -> b(202)/1, BodyDelay203/1
  b(202)/1 -> BodyLSum202/1
  BodyLSum202/1 -> BodyLSum203/2
  BodyDelay203/1 -> b(203)/1, BodyDelay204/1
  b(203)/1 -> BodyLSum203/1
  BodyLSum203/1 -> BodyLSum204/2
  BodyDelay204/1 -> b(204)/1, BodyDelay205/1
  b(204)/1 -> BodyLSum204/1
  BodyLSum204/1 -> BodyLSum205/2
  BodyDelay205/1 -> b(205)/1, BodyDelay206/1
  b(205)/1 -> BodyLSum205/1
  BodyLSum205/1 -> BodyLSum206/2
  BodyDelay206/1 -> b(206)/1, BodyDelay207/1
  b(206)/1 -> BodyLSum206/1
  BodyLSum206/1 -> BodyLSum207/2
  BodyDelay207/1 -> b(207)/1, BodyDelay208/1
  b(207)/1 -> BodyLSum207/1
  BodyLSum207/1 -> BodyLSum208/2
  BodyDelay208/1 -> b(208)/1, BodyDelay209/1
  b(208)/1 -> BodyLSum208/1
  BodyLSum208/1 -> BodyLSum209/2
  BodyDelay209/1 -> b(209)/1, BodyDelay210/1
  b(209)/1 -> BodyLSum209/1
  BodyLSum209/1 -> BodyLSum210/2
  BodyDelay210/1 -> b(210)/1, BodyDelay211/1
  b(210)/1 -> BodyLSum210/1
  BodyLSum210/1 -> BodyLSum211/2
  BodyDelay211/1 -> b(211)/1, BodyDelay212/1
  b(211)/1 -> BodyLSum211/1
  BodyLSum211/1 -> BodyLSum212/2
  BodyDelay212/1 -> b(212)/1, BodyDelay213/1
  b(212)/1 -> BodyLSum212/1
  BodyLSum212/1 -> BodyLSum213/2
  BodyDelay213/1 -> b(213)/1, BodyDelay214/1
  b(213)/1 -> BodyLSum213/1
  BodyLSum213/1 -> BodyLSum214/2
  BodyDelay214/1 -> b(214)/1, BodyDelay215/1
  b(214)/1 -> BodyLSum214/1
  BodyLSum214/1 -> BodyLSum215/2
  BodyDelay215/1 -> b(215)/1, BodyDelay216/1
  b(215)/1 -> BodyLSum215/1
  BodyLSum215/1 -> BodyLSum216/2
  BodyDelay216/1 -> b(216)/1, BodyDelay217/1
  b(216)/1 -> BodyLSum216/1
  BodyLSum216/1 -> BodyLSum217/2
  BodyDelay217/1 -> b(217)/1, BodyDelay218/1
  b(217)/1 -> BodyLSum217/1
  BodyLSum217/1 -> BodyLSum218/2
  BodyDelay218/1 -> b(218)/1, BodyDelay219/1
  b(218)/1 -> BodyLSum218/1
  BodyLSum218/1 -> BodyLSum219/2
  BodyDelay219/1 -> b(219)/1, BodyDelay220/1
  b(219)/1 -> BodyLSum219/1
  BodyLSum219/1 -> BodyLSum220/2
  BodyDelay220/1 -> b(220)/1, BodyDelay221/1
  b(220)/1 -> BodyLSum220/1
  BodyLSum220/1 -> BodyLSum221/2
  BodyDelay221/1 -> b(221)/1, BodyDelay222/1
  b(221)/1 -> BodyLSum221/1
  BodyLSum221/1 -> BodyLSum222/2
  BodyDelay222/1 -> b(222)/1, BodyDelay223/1
  b(222)/1 -> BodyLSum222/1
  BodyLSum222/1 -> BodyLSum223/2
  BodyDelay223/1 -> b(223)/1, BodyDelay224/1
  b(223)/1 -> BodyLSum223/1
  BodyLSum223/1 -> BodyLSum224/2
  BodyDelay224/1 -> b(224)/1, BodyDelay225/1
  b(224)/1 -> BodyLSum224/1
  BodyLSum224/1 -> BodyLSum225/2
  BodyDelay225/1 -> b(225)/1, BodyDelay226/1
  b(225)/1 -> BodyLSum225/1
  BodyLSum225/1 -> BodyLSum226/2
  BodyDelay226/1 -> b(226)/1, BodyDelay227/1
  b(226)/1 -> BodyLSum226/1
  BodyLSum226/1 -> BodyLSum227/2
  BodyDelay227/1 -> b(227)/1, BodyDelay228/1
  b(227)/1 -> BodyLSum227/1
  BodyLSum227/1 -> BodyLSum228/2
  BodyDelay228/1 -> b(228)/1, BodyDelay229/1
  b(228)/1 -> BodyLSum228/1
  BodyLSum228/1 -> BodyLSum229/2
  BodyDelay229/1 -> b(229)/1, BodyDelay230/1
  b(229)/1 -> BodyLSum229/1
  BodyLSum229/1 -> BodyLSum230/2
  BodyDelay230/1 -> b(230)/1, BodyDelay231/1
  b(230)/1 -> BodyLSum230/1
  BodyLSum230/1 -> BodyLSum231/2
  BodyDelay231/1 -> b(231)/1, BodyDelay232/1
  b(231)/1 -> BodyLSum231/1
  BodyLSum231/1 -> BodyLSum232/2
  BodyDelay232/1 -> b(232)/1, BodyDelay233/1
  b(232)/1 -> BodyLSum232/1
  BodyLSum232/1 -> BodyLSum233/2
  BodyDelay233/1 -> b(233)/1, BodyDelay234/1
  b(233)/1 -> BodyLSum233/1
  BodyLSum233/1 -> BodyLSum234/2
  BodyDelay234/1 -> b(234)/1, BodyDelay235/1
  b(234)/1 -> BodyLSum234/1
  BodyLSum234/1 -> BodyLSum235/2
  BodyDelay235/1 -> b(235)/1, BodyDelay236/1
  b(235)/1 -> BodyLSum235/1
  BodyLSum235/1 -> BodyLSum236/2
  BodyDelay236/1 -> b(236)/1, BodyDelay237/1
  b(236)/1 -> BodyLSum236/1
  BodyLSum236/1 -> BodyLSum237/2
  BodyDelay237/1 -> b(237)/1, BodyDelay238/1
  b(237)/1 -> BodyLSum237/1
  BodyLSum237/1 -> BodyLSum238/2
  BodyDelay238/1 -> b(238)/1, BodyDelay239/1
  b(238)/1 -> BodyLSum238/1
  BodyLSum238/1 -> BodyLSum239/2
  BodyDelay239/1 -> b(239)/1, BodyDelay240/1
  b(239)/1 -> BodyLSum239/1
  BodyLSum239/1 -> BodyLSum240/2
  BodyDelay240/1 -> b(240)/1, BodyDelay241/1
  b(240)/1 -> BodyLSum240/1
  BodyLSum240/1 -> BodyLSum241/2
  BodyDelay241/1 -> b(241)/1, BodyDelay242/1
  b(241)/1 -> BodyLSum241/1
  BodyLSum241/1 -> BodyLSum242/2
  BodyDelay242/1 -> b(242)/1, BodyDelay243/1
  b(242)/1 -> BodyLSum242/1
  BodyLSum242/1 -> BodyLSum243/2
  BodyDelay243/1 -> b(243)/1, BodyDelay244/1
  b(243)/1 -> BodyLSum243/1
  BodyLSum243/1 -> BodyLSum244/2
  BodyDelay244/1 -> b(244)/1, BodyDelay245/1
  b(244)/1 -> BodyLSum244/1
  BodyLSum244/1 -> BodyLSum245/2
  BodyDelay245/1 -> b(245)/1, BodyDelay246/1
  b(245)/1 -> BodyLSum245/1
  BodyLSum245/1 -> BodyLSum246/2
  BodyDelay246/1 -> b(246)/1, BodyDelay247/1
  b(246)/1 -> BodyLSum246/1
  BodyLSum246/1 -> BodyLSum247/2
  BodyDelay247/1 -> b(247)/1, BodyDelay248/1
  b(247)/1 -> BodyLSum247/1
  BodyLSum247/1 -> BodyLSum248/2
  BodyDelay248/1 -> b(248)/1, BodyDelay249/1
  b(248)/1 -> BodyLSum248/1
  BodyLSum248/1 -> BodyLSum249/2
  BodyDelay249/1 -> b(249)/1, BodyDelay250/1
  b(249)/1 -> BodyLSum249/1
  BodyLSum249/1 -> BodyLSum250/2
  BodyDelay250/1 -> b(250)/1, BodyDelay251/1
  b(250)/1 -> BodyLSum250/1
  BodyLSum250/1 -> BodyLSum251/2
  BodyDelay251/1 -> b(251)/1, BodyDelay252/1
  b(251)/1 -> BodyLSum251/1
  BodyLSum251/1 -> BodyLSum252/2
  BodyDelay252/1 -> b(252)/1, BodyDelay253/1
  b(252)/1 -> BodyLSum252/1
  BodyLSum252/1 -> BodyLSum253/2
  BodyDelay253/1 -> b(253)/1, BodyDelay254/1
  b(253)/1 -> BodyLSum253/1
  BodyLSum253/1 -> BodyLSum254/2
  BodyDelay254/1 -> b(254)/1, BodyDelay255/1
  b(254)/1 -> BodyLSum254/1
  BodyLSum254/1 -> BodyLSum255/2
  BodyDelay255/1 -> b(255)/1, BodyDelay256/1
  b(255)/1 -> BodyLSum255/1
  BodyLSum255/1 -> BodyLSum256/2
  BodyDelay256/1 -> b(256)/1, BodyDelay257/1
  b(256)/1 -> BodyLSum256/1
  BodyLSum256/1 -> BodyLSum257/2
  BodyDelay257/1 -> b(257)/1, BodyDelay258/1
  b(257)/1 -> BodyLSum257/1
  BodyLSum257/1 -> BodyLSum258/2
  BodyDelay258/1 -> b(258)/1, BodyDelay259/1
  b(258)/1 -> BodyLSum258/1
  BodyLSum258/1 -> BodyLSum259/2
  BodyDelay259/1 -> b(259)/1, BodyDelay260/1
  b(259)/1 -> BodyLSum259/1
  BodyLSum259/1 -> BodyLSum260/2
  BodyDelay260/1 -> b(260)/1, BodyDelay261/1
  b(260)/1 -> BodyLSum260/1
  BodyLSum260/1 -> BodyLSum261/2
  BodyDelay261/1 -> b(261)/1, BodyDelay262/1
  b(261)/1 -> BodyLSum261/1
  BodyLSum261/1 -> BodyLSum262/2
  BodyDelay262/1 -> b(262)/1, BodyDelay263/1
  b(262)/1 -> BodyLSum262/1
  BodyLSum262/1 -> BodyLSum263/2
  BodyDelay263/1 -> b(263)/1, BodyDelay264/1
  b(263)/1 -> BodyLSum263/1
  BodyLSum263/1 -> BodyLSum264/2
  BodyDelay264/1 -> b(264)/1, BodyDelay265/1
  b(264)/1 -> BodyLSum264/1
  BodyLSum264/1 -> BodyLSum265/2
  BodyDelay265/1 -> b(265)/1, BodyDelay266/1
  b(265)/1 -> BodyLSum265/1
  BodyLSum265/1 -> BodyLSum266/2
  BodyDelay266/1 -> b(266)/1, BodyDelay267/1
  b(266)/1 -> BodyLSum266/1
  BodyLSum266/1 -> BodyLSum267/2
  BodyDelay267/1 -> b(267)/1, BodyDelay268/1
  b(267)/1 -> BodyLSum267/1
  BodyLSum267/1 -> BodyLSum268/2
  BodyDelay268/1 -> b(268)/1, BodyDelay269/1
  b(268)/1 -> BodyLSum268/1
  BodyLSum268/1 -> BodyLSum269/2
  BodyDelay269/1 -> b(269)/1, BodyDelay270/1
  b(269)/1 -> BodyLSum269/1
  BodyLSum269/1 -> BodyLSum270/2
  BodyDelay270/1 -> b(270)/1, BodyDelay271/1
  b(270)/1 -> BodyLSum270/1
  BodyLSum270/1 -> BodyLSum271/2
  BodyDelay271/1 -> b(271)/1, BodyDelay272/1
  b(271)/1 -> BodyLSum271/1
  BodyLSum271/1 -> BodyLSum272/2
  BodyDelay272/1 -> b(272)/1, BodyDelay273/1
  b(272)/1 -> BodyLSum272/1
  BodyLSum272/1 -> BodyLSum273/2
  BodyDelay273/1 -> b(273)/1, BodyDelay274/1
  b(273)/1 -> BodyLSum273/1
  BodyLSum273/1 -> BodyLSum274/2
  BodyDelay274/1 -> b(274)/1, BodyDelay275/1
  b(274)/1 -> BodyLSum274/1
  BodyLSum274/1 -> BodyLSum275/2
  BodyDelay275/1 -> b(275)/1, BodyDelay276/1
  b(275)/1 -> BodyLSum275/1
  BodyLSum275/1 -> BodyLSum276/2
  BodyDelay276/1 -> b(276)/1, BodyDelay277/1
  b(276)/1 -> BodyLSum276/1
  BodyLSum276/1 -> BodyLSum277/2
  BodyDelay277/1 -> b(277)/1, BodyDelay278/1
  b(277)/1 -> BodyLSum277/1
  BodyLSum277/1 -> BodyLSum278/2
  BodyDelay278/1 -> b(278)/1, BodyDelay279/1
  b(278)/1 -> BodyLSum278/1
  BodyLSum278/1 -> BodyLSum279/2
  BodyDelay279/1 -> b(279)/1, BodyDelay280/1
  b(279)/1 -> BodyLSum279/1
  BodyLSum279/1 -> BodyLSum280/2
  BodyDelay280/1 -> b(280)/1, BodyDelay281/1
  b(280)/1 -> BodyLSum280/1
  BodyLSum280/1 -> BodyLSum281/2
  BodyDelay281/1 -> b(281)/1, BodyDelay282/1
  b(281)/1 -> BodyLSum281/1
  BodyLSum281/1 -> BodyLSum282/2
  BodyDelay282/1 -> b(282)/1, BodyDelay283/1
  b(282)/1 -> BodyLSum282/1
  BodyLSum282/1 -> BodyLSum283/2
  BodyDelay283/1 -> b(283)/1, BodyDelay284/1
  b(283)/1 -> BodyLSum283/1
  BodyLSum283/1 -> BodyLSum284/2
  BodyDelay284/1 -> b(284)/1, BodyDelay285/1
  b(284)/1 -> BodyLSum284/1
  BodyLSum284/1 -> BodyLSum285/2
  BodyDelay285/1 -> b(285)/1, BodyDelay286/1
  b(285)/1 -> BodyLSum285/1
  BodyLSum285/1 -> BodyLSum286/2
  BodyDelay286/1 -> b(286)/1, BodyDelay287/1
  b(286)/1 -> BodyLSum286/1
  BodyLSum286/1 -> BodyLSum287/2
  BodyDelay287/1 -> b(287)/1, BodyDelay288/1
  b(287)/1 -> BodyLSum287/1
  BodyLSum287/1 -> BodyLSum288/2
  BodyDelay288/1 -> b(288)/1, BodyDelay289/1
  b(288)/1 -> BodyLSum288/1
  BodyLSum288/1 -> BodyLSum289/2
  BodyDelay289/1 -> b(289)/1, BodyDelay290/1
  b(289)/1 -> BodyLSum289/1
  BodyLSum289/1 -> BodyLSum290/2
  BodyDelay290/1 -> b(290)/1, BodyDelay291/1
  b(290)/1 -> BodyLSum290/1
  BodyLSum290/1 -> BodyLSum291/2
  BodyDelay291/1 -> b(291)/1, BodyDelay292/1
  b(291)/1 -> BodyLSum291/1
  BodyLSum291/1 -> BodyLSum292/2
  BodyDelay292/1 -> b(292)/1, BodyDelay293/1
  b(292)/1 -> BodyLSum292/1
  BodyLSum292/1 -> BodyLSum293/2
  BodyDelay293/1 -> b(293)/1, BodyDelay294/1
  b(293)/1 -> BodyLSum293/1
  BodyLSum293/1 -> BodyLSum294/2
  BodyDelay294/1 -> b(294)/1, BodyDelay295/1
  b(294)/1 -> BodyLSum294/1
  BodyLSum294/1 -> BodyLSum295/2
  BodyDelay295/1 -> b(295)/1, BodyDelay296/1
  b(295)/1 -> BodyLSum295/1
  BodyLSum295/1 -> BodyLSum296/2
  BodyDelay296/1 -> b(296)/1, BodyDelay297/1
  b(296)/1 -> BodyLSum296/1
  BodyLSum296/1 -> BodyLSum297/2
  BodyDelay297/1 -> b(297)/1, BodyDelay298/1
  b(297)/1 -> BodyLSum297/1
  BodyLSum297/1 -> BodyLSum298/2
  BodyDelay298/1 -> b(298)/1, BodyDelay299/1
  b(298)/1 -> BodyLSum298/1
  BodyLSum298/1 -> BodyLSum299/2
  BodyDelay299/1 -> b(299)/1, BodyDelay300/1
  b(299)/1 -> BodyLSum299/1
  BodyLSum299/1 -> BodyLSum300/2
  BodyDelay300/1 -> b(300)/1, BodyDelay301/1
  b(300)/1 -> BodyLSum300/1
  BodyLSum300/1 -> BodyLSum301/2
  BodyDelay301/1 -> b(301)/1, BodyDelay302/1
  b(301)/1 -> BodyLSum301/1
  BodyLSum301/1 -> BodyLSum302/2
  BodyDelay302/1 -> b(302)/1, BodyDelay303/1
  b(302)/1 -> BodyLSum302/1
  BodyLSum302/1 -> BodyLSum303/2
  BodyDelay303/1 -> b(303)/1, BodyDelay304/1
  b(303)/1 -> BodyLSum303/1
  BodyLSum303/1 -> BodyLSum304/2
  BodyDelay304/1 -> b(304)/1, BodyDelay305/1
  b(304)/1 -> BodyLSum304/1
  BodyLSum304/1 -> BodyLSum305/2
  BodyDelay305/1 -> b(305)/1, BodyDelay306/1
  b(305)/1 -> BodyLSum305/1
  BodyLSum305/1 -> BodyLSum306/2
  BodyDelay306/1 -> b(306)/1, BodyDelay307/1
  b(306)/1 -> BodyLSum306/1
  BodyLSum306/1 -> BodyLSum307/2
  BodyDelay307/1 -> b(307)/1, BodyDelay308/1
  b(307)/1 -> BodyLSum307/1
  BodyLSum307/1 -> BodyLSum308/2
  BodyDelay308/1 -> b(308)/1, BodyDelay309/1
  b(308)/1 -> BodyLSum308/1
  BodyLSum308/1 -> BodyLSum309/2
  BodyDelay309/1 -> b(309)/1, BodyDelay310/1
  b(309)/1 -> BodyLSum309/1
  BodyLSum309/1 -> BodyLSum310/2
  BodyDelay310/1 -> b(310)/1, BodyDelay311/1
  b(310)/1 -> BodyLSum310/1
  BodyLSum310/1 -> BodyLSum311/2
  BodyDelay311/1 -> b(311)/1, BodyDelay312/1
  b(311)/1 -> BodyLSum311/1
  BodyLSum311/1 -> BodyLSum312/2
  BodyDelay312/1 -> b(312)/1, BodyDelay313/1
  b(312)/1 -> BodyLSum312/1
  BodyLSum312/1 -> BodyLSum313/2
  BodyDelay313/1 -> b(313)/1, BodyDelay314/1
  b(313)/1 -> BodyLSum313/1
  BodyLSum313/1 -> BodyLSum314/2
  BodyDelay314/1 -> b(314)/1, BodyDelay315/1
  b(314)/1 -> BodyLSum314/1
  BodyLSum314/1 -> BodyLSum315/2
  BodyDelay315/1 -> b(315)/1, BodyDelay316/1
  b(315)/1 -> BodyLSum315/1
  BodyLSum315/1 -> BodyLSum316/2
  BodyDelay316/1 -> b(316)/1, BodyDelay317/1
  b(316)/1 -> BodyLSum316/1
  BodyLSum316/1 -> BodyLSum317/2
  BodyDelay317/1 -> b(317)/1, BodyDelay318/1
  b(317)/1 -> BodyLSum317/1
  BodyLSum317/1 -> BodyLSum318/2
  BodyDelay318/1 -> b(318)/1, BodyDelay319/1
  b(318)/1 -> BodyLSum318/1
  BodyLSum318/1 -> BodyLSum319/2
  BodyDelay319/1 -> b(319)/1, BodyDelay320/1
  b(319)/1 -> BodyLSum319/1
  BodyLSum319/1 -> BodyLSum320/2
  BodyDelay320/1 -> b(320)/1, BodyDelay321/1
  b(320)/1 -> BodyLSum320/1
  BodyLSum320/1 -> BodyLSum321/2
  BodyDelay321/1 -> b(321)/1, BodyDelay322/1
  b(321)/1 -> BodyLSum321/1
  BodyLSum321/1 -> BodyLSum322/2
  BodyDelay322/1 -> b(322)/1, BodyDelay323/1
  b(322)/1 -> BodyLSum322/1
  BodyLSum322/1 -> BodyLSum323/2
  BodyDelay323/1 -> b(323)/1, BodyDelay324/1
  b(323)/1 -> BodyLSum323/1
  BodyLSum323/1 -> BodyLSum324/2
  BodyDelay324/1 -> b(324)/1, BodyDelay325/1
  b(324)/1 -> BodyLSum324/1
  BodyLSum324/1 -> BodyLSum325/2
  BodyDelay325/1 -> b(325)/1, BodyDelay326/1
  b(325)/1 -> BodyLSum325/1
  BodyLSum325/1 -> BodyLSum326/2
  BodyDelay326/1 -> b(326)/1, BodyDelay327/1
  b(326)/1 -> BodyLSum326/1
  BodyLSum326/1 -> BodyLSum327/2
  BodyDelay327/1 -> b(327)/1, BodyDelay328/1
  b(327)/1 -> BodyLSum327/1
  BodyLSum327/1 -> BodyLSum328/2
  BodyDelay328/1 -> b(328)/1, BodyDelay329/1
  b(328)/1 -> BodyLSum328/1
  BodyLSum328/1 -> BodyLSum329/2
  BodyDelay329/1 -> b(329)/1, BodyDelay330/1
  b(329)/1 -> BodyLSum329/1
  BodyLSum329/1 -> BodyLSum330/2
  BodyDelay330/1 -> b(330)/1, BodyDelay331/1
  b(330)/1 -> BodyLSum330/1
  BodyLSum330/1 -> BodyLSum331/2
  BodyDelay331/1 -> b(331)/1, BodyDelay332/1
  b(331)/1 -> BodyLSum331/1
  BodyLSum331/1 -> BodyLSum332/2
  BodyDelay332/1 -> b(332)/1, BodyDelay333/1
  b(332)/1 -> BodyLSum332/1
  BodyLSum332/1 -> BodyLSum333/2
  BodyDelay333/1 -> b(333)/1, BodyDelay334/1
  b(333)/1 -> BodyLSum333/1
  BodyLSum333/1 -> BodyLSum334/2
  BodyDelay334/1 -> b(334)/1, BodyDelay335/1
  b(334)/1 -> BodyLSum334/1
  BodyLSum334/1 -> BodyLSum335/2
  BodyDelay335/1 -> b(335)/1, BodyDelay336/1
  b(335)/1 -> BodyLSum335/1
  BodyLSum335/1 -> BodyLSum336/2
  BodyDelay336/1 -> b(336)/1, BodyDelay337/1
  b(336)/1 -> BodyLSum336/1
  BodyLSum336/1 -> BodyLSum337/2
  BodyDelay337/1 -> b(337)/1, BodyDelay338/1
  b(337)/1 -> BodyLSum337/1
  BodyLSum337/1 -> BodyLSum338/2
  BodyDelay338/1 -> b(338)/1, BodyDelay339/1
  b(338)/1 -> BodyLSum338/1
  BodyLSum338/1 -> BodyLSum339/2
  BodyDelay339/1 -> b(339)/1, BodyDelay340/1
  b(339)/1 -> BodyLSum339/1
  BodyLSum339/1 -> BodyLSum340/2
  BodyDelay340/1 -> b(340)/1, BodyDelay341/1
  b(340)/1 -> BodyLSum340/1
  BodyLSum340/1 -> BodyLSum341/2
  BodyDelay341/1 -> b(341)/1, BodyDelay342/1
  b(341)/1 -> BodyLSum341/1
  BodyLSum341/1 -> BodyLSum342/2
  BodyDelay342/1 -> b(342)/1, BodyDelay343/1
  b(342)/1 -> BodyLSum342/1
  BodyLSum342/1 -> BodyLSum343/2
  BodyDelay343/1 -> b(343)/1, BodyDelay344/1
  b(343)/1 -> BodyLSum343/1
  BodyLSum343/1 -> BodyLSum344/2
  BodyDelay344/1 -> b(344)/1, BodyDelay345/1
  b(344)/1 -> BodyLSum344/1
  BodyLSum344/1 -> BodyLSum345/2
  BodyDelay345/1 -> b(345)/1, BodyDelay346/1
  b(345)/1 -> BodyLSum345/1
  BodyLSum345/1 -> BodyLSum346/2
  BodyDelay346/1 -> b(346)/1, BodyDelay347/1
  b(346)/1 -> BodyLSum346/1
  BodyLSum346/1 -> BodyLSum347/2
  BodyDelay347/1 -> b(347)/1, BodyDelay348/1
  b(347)/1 -> BodyLSum347/1
  BodyLSum347/1 -> BodyLSum348/2
  BodyDelay348/1 -> b(348)/1, BodyDelay349/1
  b(348)/1 -> BodyLSum348/1
  BodyLSum348/1 -> BodyLSum349/2
  BodyDelay349/1 -> b(349)/1, BodyDelay350/1
  b(349)/1 -> BodyLSum349/1
  BodyLSum349/1 -> BodyLSum350/2
  BodyDelay350/1 -> b(350)/1, BodyDelay351/1
  b(350)/1 -> BodyLSum350/1
  BodyLSum350/1 -> BodyLSum351/2
  BodyDelay351/1 -> b(351)/1, BodyDelay352/1
  b(351)/1 -> BodyLSum351/1
  BodyLSum351/1 -> BodyLSum352/2
  BodyDelay352/1 -> b(352)/1, BodyDelay353/1
  b(352)/1 -> BodyLSum352/1
  BodyLSum352/1 -> BodyLSum353/2
  BodyDelay353/1 -> b(353)/1, BodyDelay354/1
  b(353)/1 -> BodyLSum353/1
  BodyLSum353/1 -> BodyLSum354/2
  BodyDelay354/1 -> b(354)/1, BodyDelay355/1
  b(354)/1 -> BodyLSum354/1
  BodyLSum354/1 -> BodyLSum355/2
  BodyDelay355/1 -> b(355)/1, BodyDelay356/1
  b(355)/1 -> BodyLSum355/1
  BodyLSum355/1 -> BodyLSum356/2
  BodyDelay356/1 -> b(356)/1, BodyDelay357/1
  b(356)/1 -> BodyLSum356/1
  BodyLSum356/1 -> BodyLSum357/2
  BodyDelay357/1 -> b(357)/1, BodyDelay358/1
  b(357)/1 -> BodyLSum357/1
  BodyLSum357/1 -> BodyLSum358/2
  BodyDelay358/1 -> b(358)/1, BodyDelay359/1
  b(358)/1 -> BodyLSum358/1
  BodyLSum358/1 -> BodyLSum359/2
  BodyDelay359/1 -> b(359)/1, BodyDelay360/1
  b(359)/1 -> BodyLSum359/1
  BodyLSum359/1 -> BodyLSum360/2
  BodyDelay360/1 -> b(360)/1, BodyDelay361/1
  b(360)/1 -> BodyLSum360/1
  BodyLSum360/1 -> BodyLSum361/2
  BodyDelay361/1 -> b(361)/1, BodyDelay362/1
  b(361)/1 -> BodyLSum361/1
  BodyLSum361/1 -> BodyLSum362/2
  BodyDelay362/1 -> b(362)/1, BodyDelay363/1
  b(362)/1 -> BodyLSum362/1
  BodyLSum362/1 -> BodyLSum363/2
  BodyDelay363/1 -> b(363)/1, BodyDelay364/1
  b(363)/1 -> BodyLSum363/1
  BodyLSum363/1 -> BodyLSum364/2
  BodyDelay364/1 -> b(364)/1, BodyDelay365/1
  b(364)/1 -> BodyLSum364/1
  BodyLSum364/1 -> BodyLSum365/2
  BodyDelay365/1 -> b(365)/1, BodyDelay366/1
  b(365)/1 -> BodyLSum365/1
  BodyLSum365/1 -> BodyLSum366/2
  BodyDelay366/1 -> b(366)/1, BodyDelay367/1
  b(366)/1 -> BodyLSum366/1
  BodyLSum366/1 -> BodyLSum367/2
  BodyDelay367/1 -> b(367)/1, BodyDelay368/1
  b(367)/1 -> BodyLSum367/1
  BodyLSum367/1 -> BodyLSum368/2
  BodyDelay368/1 -> b(368)/1, BodyDelay369/1
  b(368)/1 -> BodyLSum368/1
  BodyLSum368/1 -> BodyLSum369/2
  BodyDelay369/1 -> b(369)/1, BodyDelay370/1
  b(369)/1 -> BodyLSum369/1
  BodyLSum369/1 -> BodyLSum370/2
  BodyDelay370/1 -> b(370)/1, BodyDelay371/1
  b(370)/1 -> BodyLSum370/1
  BodyLSum370/1 -> BodyLSum371/2
  BodyDelay371/1 -> b(371)/1, BodyDelay372/1
  b(371)/1 -> BodyLSum371/1
  BodyLSum371/1 -> BodyLSum372/2
  BodyDelay372/1 -> b(372)/1, BodyDelay373/1
  b(372)/1 -> BodyLSum372/1
  BodyLSum372/1 -> BodyLSum373/2
  BodyDelay373/1 -> b(373)/1, BodyDelay374/1
  b(373)/1 -> BodyLSum373/1
  BodyLSum373/1 -> BodyLSum374/2
  BodyDelay374/1 -> b(374)/1, BodyDelay375/1
  b(374)/1 -> BodyLSum374/1
  BodyLSum374/1 -> BodyLSum375/2
  BodyDelay375/1 -> b(375)/1, BodyDelay376/1
  b(375)/1 -> BodyLSum375/1
  BodyLSum375/1 -> BodyLSum376/2
  BodyDelay376/1 -> b(376)/1, BodyDelay377/1
  b(376)/1 -> BodyLSum376/1
  BodyLSum376/1 -> BodyLSum377/2
  BodyDelay377/1 -> b(377)/1, BodyDelay378/1
  b(377)/1 -> BodyLSum377/1
  BodyLSum377/1 -> BodyLSum378/2
  BodyDelay378/1 -> b(378)/1, BodyDelay379/1
  b(378)/1 -> BodyLSum378/1
  BodyLSum378/1 -> BodyLSum379/2
  BodyDelay379/1 -> b(379)/1, BodyDelay380/1
  b(379)/1 -> BodyLSum379/1
  BodyLSum379/1 -> BodyLSum380/2
  BodyDelay380/1 -> b(380)/1, BodyDelay381/1
  b(380)/1 -> BodyLSum380/1
  BodyLSum380/1 -> BodyLSum381/2
  BodyDelay381/1 -> b(381)/1, BodyDelay382/1
  b(381)/1 -> BodyLSum381/1
  BodyLSum381/1 -> BodyLSum382/2
  BodyDelay382/1 -> b(382)/1, BodyDelay383/1
  b(382)/1 -> BodyLSum382/1
  BodyLSum382/1 -> BodyLSum383/2
  BodyDelay383/1 -> b(383)/1, BodyDelay384/1
  b(383)/1 -> BodyLSum383/1
  BodyLSum383/1 -> BodyLSum384/2
  BodyDelay384/1 -> b(384)/1, BodyDelay385/1
  b(384)/1 -> BodyLSum384/1
  BodyLSum384/1 -> BodyLSum385/2
  BodyDelay385/1 -> b(385)/1, BodyDelay386/1
  b(385)/1 -> BodyLSum385/1
  BodyLSum385/1 -> BodyLSum386/2
  BodyDelay386/1 -> b(386)/1, BodyDelay387/1
  b(386)/1 -> BodyLSum386/1
  BodyLSum386/1 -> BodyLSum387/2
  BodyDelay387/1 -> b(387)/1, BodyDelay388/1
  b(387)/1 -> BodyLSum387/1
  BodyLSum387/1 -> BodyLSum388/2
  BodyDelay388/1 -> b(388)/1, BodyDelay389/1
  b(388)/1 -> BodyLSum388/1
  BodyLSum388/1 -> BodyLSum389/2
  BodyDelay389/1 -> b(389)/1, BodyDelay390/1
  b(389)/1 -> BodyLSum389/1
  BodyLSum389/1 -> BodyLSum390/2
  BodyDelay390/1 -> b(390)/1, BodyDelay391/1
  b(390)/1 -> BodyLSum390/1
  BodyLSum390/1 -> BodyLSum391/2
  BodyDelay391/1 -> b(391)/1, BodyDelay392/1
  b(391)/1 -> BodyLSum391/1
  BodyLSum391/1 -> BodyLSum392/2
  BodyDelay392/1 -> b(392)/1, BodyDelay393/1
  b(392)/1 -> BodyLSum392/1
  BodyLSum392/1 -> BodyLSum393/2
  BodyDelay393/1 -> b(393)/1, BodyDelay394/1
  b(393)/1 -> BodyLSum393/1
  BodyLSum393/1 -> BodyLSum394/2
  BodyDelay394/1 -> b(394)/1, BodyDelay395/1
  b(394)/1 -> BodyLSum394/1
  BodyLSum394/1 -> BodyLSum395/2
  BodyDelay395/1 -> b(395)/1, BodyDelay396/1
  b(395)/1 -> BodyLSum395/1
  BodyLSum395/1 -> BodyLSum396/2
  BodyDelay396/1 -> b(396)/1, BodyDelay397/1
  b(396)/1 -> BodyLSum396/1
  BodyLSum396/1 -> BodyLSum397/2
  BodyDelay397/1 -> b(397)/1, BodyDelay398/1
  b(397)/1 -> BodyLSum397/1
  BodyLSum397/1 -> BodyLSum398/2
  BodyDelay398/1 -> b(398)/1, BodyDelay399/1
  b(398)/1 -> BodyLSum398/1
  BodyLSum398/1 -> BodyLSum399/2
  BodyDelay399/1 -> b(399)/1, BodyDelay400/1
  b(399)/1 -> BodyLSum399/1
  BodyLSum399/1 -> BodyLSum400/2
  BodyDelay400/1 -> b(400)/1, BodyDelay401/1
  b(400)/1 -> BodyLSum400/1
  BodyLSum400/1 -> BodyLSum401/2
  BodyDelay401/1 -> b(401)/1, BodyDelay402/1
  b(401)/1 -> BodyLSum401/1
  BodyLSum401/1 -> BodyLSum402/2
  BodyDelay402/1 -> b(402)/1, BodyDelay403/1
  b(402)/1 -> BodyLSum402/1
  BodyLSum402/1 -> BodyLSum403/2
  BodyDelay403/1 -> b(403)/1, BodyDelay404/1
  b(403)/1 -> BodyLSum403/1
  BodyLSum403/1 -> BodyLSum404/2
  BodyDelay404/1 -> b(404)/1, BodyDelay405/1
  b(404)/1 -> BodyLSum404/1
  BodyLSum404/1 -> BodyLSum405/2
  BodyDelay405/1 -> b(405)/1, BodyDelay406/1
  b(405)/1 -> BodyLSum405/1
  BodyLSum405/1 -> BodyLSum406/2
  BodyDelay406/1 -> b(406)/1, BodyDelay407/1
  b(406)/1 -> BodyLSum406/1
  BodyLSum406/1 -> BodyLSum407/2
  BodyDelay407/1 -> b(407)/1, BodyDelay408/1
  b(407)/1 -> BodyLSum407/1
  BodyLSum407/1 -> BodyLSum408/2
  BodyDelay408/1 -> b(408)/1, BodyDelay409/1
  b(408)/1 -> BodyLSum408/1
  BodyLSum408/1 -> BodyLSum409/2
  BodyDelay409/1 -> b(409)/1, BodyDelay410/1
  b(409)/1 -> BodyLSum409/1
  BodyLSum409/1 -> BodyLSum410/2
  BodyDelay410/1 -> b(410)/1, BodyDelay411/1
  b(410)/1 -> BodyLSum410/1
  BodyLSum410/1 -> BodyLSum411/2
  BodyDelay411/1 -> b(411)/1, BodyDelay412/1
  b(411)/1 -> BodyLSum411/1
  BodyLSum411/1 -> BodyLSum412/2
  BodyDelay412/1 -> b(412)/1, BodyDelay413/1
  b(412)/1 -> BodyLSum412/1
  BodyLSum412/1 -> BodyLSum413/2
  BodyDelay413/1 -> b(413)/1, BodyDelay414/1
  b(413)/1 -> BodyLSum413/1
  BodyLSum413/1 -> BodyLSum414/2
  BodyDelay414/1 -> b(414)/1, BodyDelay415/1
  b(414)/1 -> BodyLSum414/1
  BodyLSum414/1 -> BodyLSum415/2
  BodyDelay415/1 -> b(415)/1, BodyDelay416/1
  b(415)/1 -> BodyLSum415/1
  BodyLSum415/1 -> BodyLSum416/2
  BodyDelay416/1 -> b(416)/1, BodyDelay417/1
  b(416)/1 -> BodyLSum416/1
  BodyLSum416/1 -> BodyLSum417/2
  BodyDelay417/1 -> b(417)/1, BodyDelay418/1
  b(417)/1 -> BodyLSum417/1
  BodyLSum417/1 -> BodyLSum418/2
  BodyDelay418/1 -> b(418)/1, BodyDelay419/1
  b(418)/1 -> BodyLSum418/1
  BodyLSum418/1 -> BodyLSum419/2
  BodyDelay419/1 -> b(419)/1, BodyDelay420/1
  b(419)/1 -> BodyLSum419/1
  BodyLSum419/1 -> BodyLSum420/2
  BodyDelay420/1 -> b(420)/1, BodyDelay421/1
  b(420)/1 -> BodyLSum420/1
  BodyLSum420/1 -> BodyLSum421/2
  BodyDelay421/1 -> b(421)/1, BodyDelay422/1
  b(421)/1 -> BodyLSum421/1
  BodyLSum421/1 -> BodyLSum422/2
  BodyDelay422/1 -> b(422)/1, BodyDelay423/1
  b(422)/1 -> BodyLSum422/1
  BodyLSum422/1 -> BodyLSum423/2
  BodyDelay423/1 -> b(423)/1, BodyDelay424/1
  b(423)/1 -> BodyLSum423/1
  BodyLSum423/1 -> BodyLSum424/2
  BodyDelay424/1 -> b(424)/1, BodyDelay425/1
  b(424)/1 -> BodyLSum424/1
  BodyLSum424/1 -> BodyLSum425/2
  BodyDelay425/1 -> b(425)/1, BodyDelay426/1
  b(425)/1 -> BodyLSum425/1
  BodyLSum425/1 -> BodyLSum426/2
  BodyDelay426/1 -> b(426)/1, BodyDelay427/1
  b(426)/1 -> BodyLSum426/1
  BodyLSum426/1 -> BodyLSum427/2
  BodyDelay427/1 -> b(427)/1, BodyDelay428/1
  b(427)/1 -> BodyLSum427/1
  BodyLSum427/1 -> BodyLSum428/2
  BodyDelay428/1 -> b(428)/1, BodyDelay429/1
  b(428)/1 -> BodyLSum428/1
  BodyLSum428/1 -> BodyLSum429/2
  BodyDelay429/1 -> b(429)/1, BodyDelay430/1
  b(429)/1 -> BodyLSum429/1
  BodyLSum429/1 -> BodyLSum430/2
  BodyDelay430/1 -> b(430)/1, BodyDelay431/1
  b(430)/1 -> BodyLSum430/1
  BodyLSum430/1 -> BodyLSum431/2
  BodyDelay431/1 -> b(431)/1, BodyDelay432/1
  b(431)/1 -> BodyLSum431/1
  BodyLSum431/1 -> BodyLSum432/2
  BodyDelay432/1 -> b(432)/1, BodyDelay433/1
  b(432)/1 -> BodyLSum432/1
  BodyLSum432/1 -> BodyLSum433/2
  BodyDelay433/1 -> b(433)/1, BodyDelay434/1
  b(433)/1 -> BodyLSum433/1
  BodyLSum433/1 -> BodyLSum434/2
  BodyDelay434/1 -> b(434)/1, BodyDelay435/1
  b(434)/1 -> BodyLSum434/1
  BodyLSum434/1 -> BodyLSum435/2
  BodyDelay435/1 -> b(435)/1, BodyDelay436/1
  b(435)/1 -> BodyLSum435/1
  BodyLSum435/1 -> BodyLSum436/2
  BodyDelay436/1 -> b(436)/1, BodyDelay437/1
  b(436)/1 -> BodyLSum436/1
  BodyLSum436/1 -> BodyLSum437/2
  BodyDelay437/1 -> b(437)/1, BodyDelay438/1
  b(437)/1 -> BodyLSum437/1
  BodyLSum437/1 -> BodyLSum438/2
  BodyDelay438/1 -> b(438)/1, BodyDelay439/1
  b(438)/1 -> BodyLSum438/1
  BodyLSum438/1 -> BodyLSum439/2
  BodyDelay439/1 -> b(439)/1, BodyDelay440/1
  b(439)/1 -> BodyLSum439/1
  BodyLSum439/1 -> BodyLSum440/2
  BodyDelay440/1 -> b(440)/1, BodyDelay441/1
  b(440)/1 -> BodyLSum440/1
  BodyLSum440/1 -> BodyLSum441/2
  BodyDelay441/1 -> b(441)/1, BodyDelay442/1
  b(441)/1 -> BodyLSum441/1
  BodyLSum441/1 -> BodyLSum442/2
  BodyDelay442/1 -> b(442)/1, BodyDelay443/1
  b(442)/1 -> BodyLSum442/1
  BodyLSum442/1 -> BodyLSum443/2
  BodyDelay443/1 -> b(443)/1, BodyDelay444/1
  b(443)/1 -> BodyLSum443/1
  BodyLSum443/1 -> BodyLSum444/2
  BodyDelay444/1 -> b(444)/1, BodyDelay445/1
  b(444)/1 -> BodyLSum444/1
  BodyLSum444/1 -> BodyLSum445/2
  BodyDelay445/1 -> b(445)/1, BodyDelay446/1
  b(445)/1 -> BodyLSum445/1
  BodyLSum445/1 -> BodyLSum446/2
  BodyDelay446/1 -> b(446)/1, BodyDelay447/1
  b(446)/1 -> BodyLSum446/1
  BodyLSum446/1 -> BodyLSum447/2
  BodyDelay447/1 -> b(447)/1, BodyDelay448/1
  b(447)/1 -> BodyLSum447/1
  BodyLSum447/1 -> BodyLSum448/2
  BodyDelay448/1 -> b(448)/1, BodyDelay449/1
  b(448)/1 -> BodyLSum448/1
  BodyLSum448/1 -> BodyLSum449/2
  BodyDelay449/1 -> b(449)/1, BodyDelay450/1
  b(449)/1 -> BodyLSum449/1
  BodyLSum449/1 -> BodyLSum450/2
  BodyDelay450/1 -> b(450)/1, BodyDelay451/1
  b(450)/1 -> BodyLSum450/1
  BodyLSum450/1 -> BodyLSum451/2
  BodyDelay451/1 -> b(451)/1, BodyDelay452/1
  b(451)/1 -> BodyLSum451/1
  BodyLSum451/1 -> BodyLSum452/2
  BodyDelay452/1 -> b(452)/1, BodyDelay453/1
  b(452)/1 -> BodyLSum452/1
  BodyLSum452/1 -> BodyLSum453/2
  BodyDelay453/1 -> b(453)/1, BodyDelay454/1
  b(453)/1 -> BodyLSum453/1
  BodyLSum453/1 -> BodyLSum454/2
  BodyDelay454/1 -> b(454)/1, BodyDelay455/1
  b(454)/1 -> BodyLSum454/1
  BodyLSum454/1 -> BodyLSum455/2
  BodyDelay455/1 -> b(455)/1, BodyDelay456/1
  b(455)/1 -> BodyLSum455/1
  BodyLSum455/1 -> BodyLSum456/2
  BodyDelay456/1 -> b(456)/1, BodyDelay457/1
  b(456)/1 -> BodyLSum456/1
  BodyLSum456/1 -> BodyLSum457/2
  BodyDelay457/1 -> b(457)/1, BodyDelay458/1
  b(457)/1 -> BodyLSum457/1
  BodyLSum457/1 -> BodyLSum458/2
  BodyDelay458/1 -> b(458)/1, BodyDelay459/1
  b(458)/1 -> BodyLSum458/1
  BodyLSum458/1 -> BodyLSum459/2
  BodyDelay459/1 -> b(459)/1, BodyDelay460/1
  b(459)/1 -> BodyLSum459/1
  BodyLSum459/1 -> BodyLSum460/2
  BodyDelay460/1 -> b(460)/1, BodyDelay461/1
  b(460)/1 -> BodyLSum460/1
  BodyLSum460/1 -> BodyLSum461/2
  BodyDelay461/1 -> b(461)/1, BodyDelay462/1
  b(461)/1 -> BodyLSum461/1
  BodyLSum461/1 -> BodyLSum462/2
  BodyDelay462/1 -> b(462)/1, BodyDelay463/1
  b(462)/1 -> BodyLSum462/1
  BodyLSum462/1 -> BodyLSum463/2
  BodyDelay463/1 -> b(463)/1, BodyDelay464/1
  b(463)/1 -> BodyLSum463/1
  BodyLSum463/1 -> BodyLSum464/2
  BodyDelay464/1 -> b(464)/1, BodyDelay465/1
  b(464)/1 -> BodyLSum464/1
  BodyLSum464/1 -> BodyLSum465/2
  BodyDelay465/1 -> b(465)/1, BodyDelay466/1
  b(465)/1 -> BodyLSum465/1
  BodyLSum465/1 -> BodyLSum466/2
  BodyDelay466/1 -> b(466)/1, BodyDelay467/1
  b(466)/1 -> BodyLSum466/1
  BodyLSum466/1 -> BodyLSum467/2
  BodyDelay467/1 -> b(467)/1, BodyDelay468/1
  b(467)/1 -> BodyLSum467/1
  BodyLSum467/1 -> BodyLSum468/2
  BodyDelay468/1 -> b(468)/1, BodyDelay469/1
  b(468)/1 -> BodyLSum468/1
  BodyLSum468/1 -> BodyLSum469/2
  BodyDelay469/1 -> b(469)/1, BodyDelay470/1
  b(469)/1 -> BodyLSum469/1
  BodyLSum469/1 -> BodyLSum470/2
  BodyDelay470/1 -> b(470)/1, BodyDelay471/1
  b(470)/1 -> BodyLSum470/1
  BodyLSum470/1 -> BodyLSum471/2
  BodyDelay471/1 -> b(471)/1, BodyDelay472/1
  b(471)/1 -> BodyLSum471/1
  BodyLSum471/1 -> BodyLSum472/2
  BodyDelay472/1 -> b(472)/1, BodyDelay473/1
  b(472)/1 -> BodyLSum472/1
  BodyLSum472/1 -> BodyLSum473/2
  BodyDelay473/1 -> b(473)/1, BodyDelay474/1
  b(473)/1 -> BodyLSum473/1
  BodyLSum473/1 -> BodyLSum474/2
  BodyDelay474/1 -> b(474)/1, BodyDelay475/1
  b(474)/1 -> BodyLSum474/1
  BodyLSum474/1 -> BodyLSum475/2
  BodyDelay475/1 -> b(475)/1, BodyDelay476/1
  b(475)/1 -> BodyLSum475/1
  BodyLSum475/1 -> BodyLSum476/2
  BodyDelay476/1 -> b(476)/1, BodyDelay477/1
  b(476)/1 -> BodyLSum476/1
  BodyLSum476/1 -> BodyLSum477/2
  BodyDelay477/1 -> b(477)/1, BodyDelay478/1
  b(477)/1 -> BodyLSum477/1
  BodyLSum477/1 -> BodyLSum478/2
  BodyDelay478/1 -> b(478)/1, BodyDelay479/1
  b(478)/1 -> BodyLSum478/1
  BodyLSum478/1 -> BodyLSum479/2
  BodyDelay479/1 -> b(479)/1, BodyDelay480/1
  b(479)/1 -> BodyLSum479/1
  BodyLSum479/1 -> BodyLSum480/2
  BodyDelay480/1 -> b(480)/1, BodyDelay481/1
  b(480)/1 -> BodyLSum480/1
  BodyLSum480/1 -> BodyLSum481/2
  BodyDelay481/1 -> b(481)/1, BodyDelay482/1
  b(481)/1 -> BodyLSum481/1
  BodyLSum481/1 -> BodyLSum482/2
  BodyDelay482/1 -> b(482)/1, BodyDelay483/1
  b(482)/1 -> BodyLSum482/1
  BodyLSum482/1 -> BodyLSum483/2
  BodyDelay483/1 -> b(483)/1, BodyDelay484/1
  b(483)/1 -> BodyLSum483/1
  BodyLSum483/1 -> BodyLSum484/2
  BodyDelay484/1 -> b(484)/1, BodyDelay485/1
  b(484)/1 -> BodyLSum484/1
  BodyLSum484/1 -> BodyLSum485/2
  BodyDelay485/1 -> b(485)/1, BodyDelay486/1
  b(485)/1 -> BodyLSum485/1
  BodyLSum485/1 -> BodyLSum486/2
  BodyDelay486/1 -> b(486)/1, BodyDelay487/1
  b(486)/1 -> BodyLSum486/1
  BodyLSum486/1 -> BodyLSum487/2
  BodyDelay487/1 -> b(487)/1, BodyDelay488/1
  b(487)/1 -> BodyLSum487/1
  BodyLSum487/1 -> BodyLSum488/2
  BodyDelay488/1 -> b(488)/1, BodyDelay489/1
  b(488)/1 -> BodyLSum488/1
  BodyLSum488/1 -> BodyLSum489/2
  BodyDelay489/1 -> b(489)/1, BodyDelay490/1
  b(489)/1 -> BodyLSum489/1
  BodyLSum489/1 -> BodyLSum490/2
  BodyDelay490/1 -> b(490)/1, BodyDelay491/1
  b(490)/1 -> BodyLSum490/1
  BodyLSum490/1 -> BodyLSum491/2
  BodyDelay491/1 -> b(491)/1, BodyDelay492/1
  b(491)/1 -> BodyLSum491/1
  BodyLSum491/1 -> BodyLSum492/2
  BodyDelay492/1 -> b(492)/1, BodyDelay493/1
  b(492)/1 -> BodyLSum492/1
  BodyLSum492/1 -> BodyLSum493/2
  BodyDelay493/1 -> b(493)/1, BodyDelay494/1
  b(493)/1 -> BodyLSum493/1
  BodyLSum493/1 -> BodyLSum494/2
  BodyDelay494/1 -> b(494)/1, BodyDelay495/1
  b(494)/1 -> BodyLSum494/1
  BodyLSum494/1 -> BodyLSum495/2
  BodyDelay495/1 -> b(495)/1, BodyDelay496/1
  b(495)/1 -> BodyLSum495/1
  BodyLSum495/1 -> BodyLSum496/2
  BodyDelay496/1 -> b(496)/1, BodyDelay497/1
  b(496)/1 -> BodyLSum496/1
  BodyLSum496/1 -> BodyLSum497/2
  BodyDelay497/1 -> b(497)/1, BodyDelay498/1
  b(497)/1 -> BodyLSum497/1
  BodyLSum497/1 -> BodyLSum498/2
  BodyDelay498/1 -> b(498)/1, BodyDelay499/1
  b(498)/1 -> BodyLSum498/1
  BodyLSum498/1 -> BodyLSum499/2
  BodyDelay499/1 -> b(499)/1, BodyDelay500/1
  b(499)/1 -> BodyLSum499/1
  BodyLSum499/1 -> BodyLSum500/2
  BodyDelay500/1 -> b(500)/1, BodyDelay501/1
  b(500)/1 -> BodyLSum500/1
  BodyLSum500/1 -> BodyLSum501/2
  BodyDelay501/1 -> b(501)/1, BodyDelay502/1
  b(501)/1 -> BodyLSum501/1
  BodyLSum501/1 -> BodyLSum502/2
  BodyDelay502/1 -> b(502)/1, BodyDelay503/1
  b(502)/1 -> BodyLSum502/1
  BodyLSum502/1 -> BodyLSum503/2
  BodyDelay503/1 -> b(503)/1, BodyDelay504/1
  b(503)/1 -> BodyLSum503/1
  BodyLSum503/1 -> BodyLSum504/2
  BodyDelay504/1 -> b(504)/1, BodyDelay505/1
  b(504)/1 -> BodyLSum504/1
  BodyLSum504/1 -> BodyLSum505/2
  BodyDelay505/1 -> b(505)/1, BodyDelay506/1
  b(505)/1 -> BodyLSum505/1
  BodyLSum505/1 -> BodyLSum506/2
  BodyDelay506/1 -> b(506)/1, BodyDelay507/1
  b(506)/1 -> BodyLSum506/1
  BodyLSum506/1 -> BodyLSum507/2
  BodyDelay507/1 -> b(507)/1, BodyDelay508/1
  b(507)/1 -> BodyLSum507/1
  BodyLSum507/1 -> BodyLSum508/2
  BodyDelay508/1 -> b(508)/1, BodyDelay509/1
  b(508)/1 -> BodyLSum508/1
  BodyLSum508/1 -> BodyLSum509/2
  BodyDelay509/1 -> b(509)/1, BodyDelay510/1
  b(509)/1 -> BodyLSum509/1
  BodyLSum509/1 -> BodyLSum510/2
  BodyDelay510/1 -> b(510)/1, BodyDelay511/1
  b(510)/1 -> BodyLSum510/1
  BodyLSum510/1 -> BodyLSum511/2
  BodyDelay511/1 -> b(511)/1, BodyDelay512/1
  b(511)/1 -> BodyLSum511/1
  BodyLSum511/1 -> BodyLSum512/2
  BodyDelay512/1 -> b(512)/1, BodyDelay513/1
  b(512)/1 -> BodyLSum512/1
  BodyLSum512/1 -> BodyLSum513/2
  BodyDelay513/1 -> b(513)/1, BodyDelay514/1
  b(513)/1 -> BodyLSum513/1
  BodyLSum513/1 -> BodyLSum514/2
  BodyDelay514/1 -> b(514)/1, BodyDelay515/1
  b(514)/1 -> BodyLSum514/1
  BodyLSum514/1 -> BodyLSum515/2
  BodyDelay515/1 -> b(515)/1, BodyDelay516/1
  b(515)/1 -> BodyLSum515/1
  BodyLSum515/1 -> BodyLSum516/2
  BodyDelay516/1 -> b(516)/1, BodyDelay517/1
  b(516)/1 -> BodyLSum516/1
  BodyLSum516/1 -> BodyLSum517/2
  BodyDelay517/1 -> b(517)/1, BodyDelay518/1
  b(517)/1 -> BodyLSum517/1
  BodyLSum517/1 -> BodyLSum518/2
  BodyDelay518/1 -> b(518)/1, BodyDelay519/1
  b(518)/1 -> BodyLSum518/1
  BodyLSum518/1 -> BodyLSum519/2
  BodyDelay519/1 -> b(519)/1, BodyDelay520/1
  b(519)/1 -> BodyLSum519/1
  BodyLSum519/1 -> BodyLSum520/2
  BodyDelay520/1 -> b(520)/1, BodyDelay521/1
  b(520)/1 -> BodyLSum520/1
  BodyLSum520/1 -> BodyLSum521/2
  BodyDelay521/1 -> b(521)/1, BodyDelay522/1
  b(521)/1 -> BodyLSum521/1
  BodyLSum521/1 -> BodyLSum522/2
  BodyDelay522/1 -> b(522)/1, BodyDelay523/1
  b(522)/1 -> BodyLSum522/1
  BodyLSum522/1 -> BodyLSum523/2
  BodyDelay523/1 -> b(523)/1, BodyDelay524/1
  b(523)/1 -> BodyLSum523/1
  BodyLSum523/1 -> BodyLSum524/2
  BodyDelay524/1 -> b(524)/1, BodyDelay525/1
  b(524)/1 -> BodyLSum524/1
  BodyLSum524/1 -> BodyLSum525/2
  BodyDelay525/1 -> b(525)/1, BodyDelay526/1
  b(525)/1 -> BodyLSum525/1
  BodyLSum525/1 -> BodyLSum526/2
  BodyDelay526/1 -> b(526)/1, BodyDelay527/1
  b(526)/1 -> BodyLSum526/1
  BodyLSum526/1 -> BodyLSum527/2
  BodyDelay527/1 -> b(527)/1, BodyDelay528/1
  b(527)/1 -> BodyLSum527/1
  BodyLSum527/1 -> BodyLSum528/1
  BodyDelay528/1 -> b(528)/1
  b(528)/1 -> BodyLSum528/2
  BodyLSum528/1 -> Output/1
